simulink model "KUKA_LBR_Simulink_model_flatness_based_control"  (R2017a)
(part 3 of 19)

  cos(q2).*cos(q3).*sin(q1)+cos(q1).*sin(q3))+sin(q1).*sin(q2).*sin(q4))+( ...
  cos(q1).*cos(q3)+(-1).*cos(q2).*sin(q1).*sin(q3)).*sin(q5))+((-1).*cos( ...
  q4).*sin(q1).*sin(q2)+(cos(q2).*cos(q3).*sin(q1)+cos(q1).*sin(q3)).*sin( ...
  q4)).*sin(q6))+(cos(q5).*(cos(q1).*cos(q3)+(-1).*cos(q2).*sin(q1).*sin( ...
  q3))+(-1).*(cos(q4).*(cos(q2).*cos(q3).*sin(q1)+cos(q1).*sin(q3))+sin( ...
  q1).*sin(q2).*sin(q4)).*sin(q5)).*sin(q7)).^2.*(cos(q7).*(cos(q5).*((-1) ...
  .*cos(q3).*sin(q1)+(-1).*cos(q1).*cos(q2).*sin(q3))+(-1).*(cos(q4).*( ...
  cos(q1).*cos(q2).*cos(q3)+(-1).*sin(q1).*sin(q3))+cos(q1).*sin(q2).*sin( ...
  q4)).*sin(q5))+(-1).*(cos(q6).*(cos(q5).*(cos(q4).*(cos(q1).*cos(q2).* ...
  cos(q3)+(-1).*sin(q1).*sin(q3))+cos(q1).*sin(q2).*sin(q4))+((-1).*cos( ...
  q3).*sin(q1)+(-1).*cos(q1).*cos(q2).*sin(q3)).*sin(q5))+((-1).*cos(q1).* ...
  cos(q4).*sin(q2)+(cos(q1).*cos(q2).*cos(q3)+(-1).*sin(q1).*sin(q3)).* ...
  sin(q4)).*sin(q6)).*sin(q7)))+(1+(cos(q7).*(cos(q6).*(cos(q5).*(cos(q4) ...
  .*(cos(q1).*cos(q2).*cos(q3)+(-1).*sin(q1).*sin(q3))+cos(q1).*sin(q2).* ...
  sin(q4))+((-1).*cos(q3).*sin(q1)+(-1).*cos(q1).*cos(q2).*sin(q3)).*sin( ...
  q5))+((-1).*cos(q1).*cos(q4).*sin(q2)+(cos(q1).*cos(q2).*cos(q3)+(-1).* ...
  sin(q1).*sin(q3)).*sin(q4)).*sin(q6))+(cos(q5).*((-1).*cos(q3).*sin(q1)+ ...
  (-1).*cos(q1).*cos(q2).*sin(q3))+(-1).*(cos(q4).*(cos(q1).*cos(q2).*cos( ...
  q3)+(-1).*sin(q1).*sin(q3))+cos(q1).*sin(q2).*sin(q4)).*sin(q5)).*sin( ...
  q7)).^(-2).*(cos(q7).*(cos(q6).*(cos(q5).*(cos(q4).*(cos(q2).*cos(q3).* ...
  sin(q1)+cos(q1).*sin(q3))+sin(q1).*sin(q2).*sin(q4))+(cos(q1).*cos(q3)+( ...
  -1).*cos(q2).*sin(q1).*sin(q3)).*sin(q5))+((-1).*cos(q4).*sin(q1).*sin( ...
  q2)+(cos(q2).*cos(q3).*sin(q1)+cos(q1).*sin(q3)).*sin(q4)).*sin(q6))+( ...
  cos(q5).*(cos(q1).*cos(q3)+(-1).*cos(q2).*sin(q1).*sin(q3))+(-1).*(cos( ...
  q4).*(cos(q2).*cos(q3).*sin(q1)+cos(q1).*sin(q3))+sin(q1).*sin(q2).*sin( ...
  q4)).*sin(q5)).*sin(q7)).^2).^(-1).*((cos(q7).*(cos(q6).*(cos(q5).*(cos( ...
  q4).*(cos(q1).*cos(q2).*cos(q3)+(-1).*sin(q1).*sin(q3))+cos(q1).*sin(q2) ...
  .*sin(q4))+((-1).*cos(q3).*sin(q1)+(-1).*cos(q1).*cos(q2).*sin(q3)).* ...
  sin(q5))+((-1).*cos(q1).*cos(q4).*sin(q2)+(cos(q1).*cos(q2).*cos(q3)+( ...
  -1).*sin(q1).*sin(q3)).*sin(q4)).*sin(q6))+(cos(q5).*((-1).*cos(q3).* ...
  sin(q1)+(-1).*cos(q1).*cos(q2).*sin(q3))+(-1).*(cos(q4).*(cos(q1).*cos( ...
  q2).*cos(q3)+(-1).*sin(q1).*sin(q3))+cos(q1).*sin(q2).*sin(q4)).*sin(q5) ...
  ).*sin(q7)).^(-1).*((-1).*cos(q7).*(cos(q6).*(cos(q5).*(cos(q4).*(cos( ...
  q2).*cos(q3).*sin(q1)+cos(q1).*sin(q3))+sin(q1).*sin(q2).*sin(q4))+(cos( ...
  q1).*cos(q3)+(-1).*cos(q2).*sin(q1).*sin(q3)).*sin(q5))+((-1).*cos(q4).* ...
  sin(q1).*sin(q2)+(cos(q2).*cos(q3).*sin(q1)+cos(q1).*sin(q3)).*sin(q4)) ...
  .*sin(q6))+(-1).*(cos(q5).*(cos(q1).*cos(q3)+(-1).*cos(q2).*sin(q1).* ...
  sin(q3))+(-1).*(cos(q4).*(cos(q2).*cos(q3).*sin(q1)+cos(q1).*sin(q3))+ ...
  sin(q1).*sin(q2).*sin(q4)).*sin(q5)).*sin(q7))+(-1).*((-1).*cos(q7).*( ...
  cos(q6).*(cos(q5).*(cos(q4).*(cos(q1).*cos(q2).*cos(q3)+(-1).*sin(q1).* ...
  sin(q3))+cos(q1).*sin(q2).*sin(q4))+((-1).*cos(q3).*sin(q1)+(-1).*cos( ...
  q1).*cos(q2).*sin(q3)).*sin(q5))+((-1).*cos(q1).*cos(q4).*sin(q2)+(cos( ...
  q1).*cos(q2).*cos(q3)+(-1).*sin(q1).*sin(q3)).*sin(q4)).*sin(q6))+(-1).* ...
  (cos(q5).*((-1).*cos(q3).*sin(q1)+(-1).*cos(q1).*cos(q2).*sin(q3))+(-1) ...
  .*(cos(q4).*(cos(q1).*cos(q2).*cos(q3)+(-1).*sin(q1).*sin(q3))+cos(q1).* ...
  sin(q2).*sin(q4)).*sin(q5)).*sin(q7)).*(cos(q7).*(cos(q6).*(cos(q5).*( ...
  cos(q4).*(cos(q1).*cos(q2).*cos(q3)+(-1).*sin(q1).*sin(q3))+cos(q1).* ...
  sin(q2).*sin(q4))+((-1).*cos(q3).*sin(q1)+(-1).*cos(q1).*cos(q2).*sin( ...
  q3)).*sin(q5))+((-1).*cos(q1).*cos(q4).*sin(q2)+(cos(q1).*cos(q2).*cos( ...
  q3)+(-1).*sin(q1).*sin(q3)).*sin(q4)).*sin(q6))+(cos(q5).*((-1).*cos(q3) ...
  .*sin(q1)+(-1).*cos(q1).*cos(q2).*sin(q3))+(-1).*(cos(q4).*(cos(q1).* ...
  cos(q2).*cos(q3)+(-1).*sin(q1).*sin(q3))+cos(q1).*sin(q2).*sin(q4)).* ...
  sin(q5)).*sin(q7)).^(-2).*(cos(q7).*(cos(q6).*(cos(q5).*(cos(q4).*(cos( ...
  q2).*cos(q3).*sin(q1)+cos(q1).*sin(q3))+sin(q1).*sin(q2).*sin(q4))+(cos( ...
  q1).*cos(q3)+(-1).*cos(q2).*sin(q1).*sin(q3)).*sin(q5))+((-1).*cos(q4).* ...
  sin(q1).*sin(q2)+(cos(q2).*cos(q3).*sin(q1)+cos(q1).*sin(q3)).*sin(q4)) ...
  .*sin(q6))+(cos(q5).*(cos(q1).*cos(q3)+(-1).*cos(q2).*sin(q1).*sin(q3))+ ...
  (-1).*(cos(q4).*(cos(q2).*cos(q3).*sin(q1)+cos(q1).*sin(q3))+sin(q1).* ...
  sin(q2).*sin(q4)).*sin(q5)).*sin(q7))+(-2).*(cos(q7).*(cos(q6).*(cos(q5) ...
  .*(cos(q4).*(cos(q1).*cos(q2).*cos(q3)+(-1).*sin(q1).*sin(q3))+cos(q1).* ...
  sin(q2).*sin(q4))+((-1).*cos(q3).*sin(q1)+(-1).*cos(q1).*cos(q2).*sin( ...
  q3)).*sin(q5))+((-1).*cos(q1).*cos(q4).*sin(q2)+(cos(q1).*cos(q2).*cos( ...
  q3)+(-1).*sin(q1).*sin(q3)).*sin(q4)).*sin(q6))+(cos(q5).*((-1).*cos(q3) ...
  .*sin(q1)+(-1).*cos(q1).*cos(q2).*sin(q3))+(-1).*(cos(q4).*(cos(q1).* ...
  cos(q2).*cos(q3)+(-1).*sin(q1).*sin(q3))+cos(q1).*sin(q2).*sin(q4)).* ...
  sin(q5)).*sin(q7)).^(-2).*(cos(q7).*(cos(q5).*(cos(q1).*cos(q3)+(-1).* ...
  cos(q2).*sin(q1).*sin(q3))+(-1).*(cos(q4).*(cos(q2).*cos(q3).*sin(q1)+ ...
  cos(q1).*sin(q3))+sin(q1).*sin(q2).*sin(q4)).*sin(q5))+(-1).*(cos(q6).*( ...
  cos(q5).*(cos(q4).*(cos(q2).*cos(q3).*sin(q1)+cos(q1).*sin(q3))+sin(q1) ...
  .*sin(q2).*sin(q4))+(cos(q1).*cos(q3)+(-1).*cos(q2).*sin(q1).*sin(q3)).* ...
  sin(q5))+((-1).*cos(q4).*sin(q1).*sin(q2)+(cos(q2).*cos(q3).*sin(q1)+ ...
  cos(q1).*sin(q3)).*sin(q4)).*sin(q6)).*sin(q7)).*(cos(q7).*(cos(q5).*(( ...
  -1).*cos(q3).*sin(q1)+(-1).*cos(q1).*cos(q2).*sin(q3))+(-1).*(cos(q4).*( ...
  cos(q1).*cos(q2).*cos(q3)+(-1).*sin(q1).*sin(q3))+cos(q1).*sin(q2).*sin( ...
  q4)).*sin(q5))+(-1).*(cos(q6).*(cos(q5).*(cos(q4).*(cos(q1).*cos(q2).* ...
  cos(q3)+(-1).*sin(q1).*sin(q3))+cos(q1).*sin(q2).*sin(q4))+((-1).*cos( ...
  q3).*sin(q1)+(-1).*cos(q1).*cos(q2).*sin(q3)).*sin(q5))+((-1).*cos(q1).* ...
  cos(q4).*sin(q2)+(cos(q1).*cos(q2).*cos(q3)+(-1).*sin(q1).*sin(q3)).* ...
  sin(q4)).*sin(q6)).*sin(q7))+2.*(cos(q7).*(cos(q6).*(cos(q5).*(cos(q4).* ...
  (cos(q1).*cos(q2).*cos(q3)+(-1).*sin(q1).*sin(q3))+cos(q1).*sin(q2).* ...
  sin(q4))+((-1).*cos(q3).*sin(q1)+(-1).*cos(q1).*cos(q2).*sin(q3)).*sin( ...
  q5))+((-1).*cos(q1).*cos(q4).*sin(q2)+(cos(q1).*cos(q2).*cos(q3)+(-1).* ...
  sin(q1).*sin(q3)).*sin(q4)).*sin(q6))+(cos(q5).*((-1).*cos(q3).*sin(q1)+ ...
  (-1).*cos(q1).*cos(q2).*sin(q3))+(-1).*(cos(q4).*(cos(q1).*cos(q2).*cos( ...
  q3)+(-1).*sin(q1).*sin(q3))+cos(q1).*sin(q2).*sin(q4)).*sin(q5)).*sin( ...
  q7)).^(-3).*(cos(q7).*(cos(q6).*(cos(q5).*(cos(q4).*(cos(q2).*cos(q3).* ...
  sin(q1)+cos(q1).*sin(q3))+sin(q1).*sin(q2).*sin(q4))+(cos(q1).*cos(q3)+( ...
  -1).*cos(q2).*sin(q1).*sin(q3)).*sin(q5))+((-1).*cos(q4).*sin(q1).*sin( ...
  q2)+(cos(q2).*cos(q3).*sin(q1)+cos(q1).*sin(q3)).*sin(q4)).*sin(q6))+( ...
  cos(q5).*(cos(q1).*cos(q3)+(-1).*cos(q2).*sin(q1).*sin(q3))+(-1).*(cos( ...
  q4).*(cos(q2).*cos(q3).*sin(q1)+cos(q1).*sin(q3))+sin(q1).*sin(q2).*sin( ...
  q4)).*sin(q5)).*sin(q7)).*(cos(q7).*(cos(q5).*((-1).*cos(q3).*sin(q1)+( ...
  -1).*cos(q1).*cos(q2).*sin(q3))+(-1).*(cos(q4).*(cos(q1).*cos(q2).*cos( ...
  q3)+(-1).*sin(q1).*sin(q3))+cos(q1).*sin(q2).*sin(q4)).*sin(q5))+(-1).*( ...
  cos(q6).*(cos(q5).*(cos(q4).*(cos(q1).*cos(q2).*cos(q3)+(-1).*sin(q1).* ...
  sin(q3))+cos(q1).*sin(q2).*sin(q4))+((-1).*cos(q3).*sin(q1)+(-1).*cos( ...
  q1).*cos(q2).*sin(q3)).*sin(q5))+((-1).*cos(q1).*cos(q4).*sin(q2)+(cos( ...
  q1).*cos(q2).*cos(q3)+(-1).*sin(q1).*sin(q3)).*sin(q4)).*sin(q6)).*sin( ...
  q7)).^2);

Jxe251 = 0;

Jxe252 = (-1).*(1+(cos(q7).*(cos(q6).*(cos(q5).*((-1).*cos(q3).*cos( ...
  q4).*sin(q2)+cos(q2).*sin(q4))+sin(q2).*sin(q3).*sin(q5))+((-1).*cos(q2) ...
  .*cos(q4)+(-1).*cos(q3).*sin(q2).*sin(q4)).*sin(q6))+(cos(q5).*sin(q2).* ...
  sin(q3)+(-1).*((-1).*cos(q3).*cos(q4).*sin(q2)+cos(q2).*sin(q4)).*sin( ...
  q5)).*sin(q7)).^2.*(((-1).*cos(q6).*((-1).*cos(q2).*cos(q4)+(-1).*cos( ...
  q3).*sin(q2).*sin(q4))+(cos(q5).*((-1).*cos(q3).*cos(q4).*sin(q2)+cos( ...
  q2).*sin(q4))+sin(q2).*sin(q3).*sin(q5)).*sin(q6)).^2+(cos(q7).*(cos(q5) ...
  .*sin(q2).*sin(q3)+(-1).*((-1).*cos(q3).*cos(q4).*sin(q2)+cos(q2).*sin( ...
  q4)).*sin(q5))+(-1).*(cos(q6).*(cos(q5).*((-1).*cos(q3).*cos(q4).*sin( ...
  q2)+cos(q2).*sin(q4))+sin(q2).*sin(q3).*sin(q5))+((-1).*cos(q2).*cos(q4) ...
  +(-1).*cos(q3).*sin(q2).*sin(q4)).*sin(q6)).*sin(q7)).^2).^(-1)).^(-2).* ...
  ((-1).*(cos(q7).*(cos(q6).*(cos(q5).*((-1).*cos(q3).*cos(q4).*sin(q2)+ ...
  cos(q2).*sin(q4))+sin(q2).*sin(q3).*sin(q5))+((-1).*cos(q2).*cos(q4)+( ...
  -1).*cos(q3).*sin(q2).*sin(q4)).*sin(q6))+(cos(q5).*sin(q2).*sin(q3)+( ...
  -1).*((-1).*cos(q3).*cos(q4).*sin(q2)+cos(q2).*sin(q4)).*sin(q5)).*sin( ...
  q7)).^2.*(2.*((-1).*cos(q6).*(cos(q4).*sin(q2)+(-1).*cos(q2).*cos(q3).* ...
  sin(q4))+(cos(q5).*((-1).*cos(q2).*cos(q3).*cos(q4)+(-1).*sin(q2).*sin( ...
  q4))+cos(q2).*sin(q3).*sin(q5)).*sin(q6)).*((-1).*cos(q6).*((-1).*cos( ...
  q2).*cos(q4)+(-1).*cos(q3).*sin(q2).*sin(q4))+(cos(q5).*((-1).*cos(q3).* ...
  cos(q4).*sin(q2)+cos(q2).*sin(q4))+sin(q2).*sin(q3).*sin(q5)).*sin(q6))+ ...
  2.*(cos(q7).*(cos(q2).*cos(q5).*sin(q3)+(-1).*((-1).*cos(q2).*cos(q3).* ...
  cos(q4)+(-1).*sin(q2).*sin(q4)).*sin(q5))+(-1).*(cos(q6).*(cos(q5).*(( ...
  -1).*cos(q2).*cos(q3).*cos(q4)+(-1).*sin(q2).*sin(q4))+cos(q2).*sin(q3) ...
  .*sin(q5))+(cos(q4).*sin(q2)+(-1).*cos(q2).*cos(q3).*sin(q4)).*sin(q6)) ...
  .*sin(q7)).*(cos(q7).*(cos(q5).*sin(q2).*sin(q3)+(-1).*((-1).*cos(q3).* ...
  cos(q4).*sin(q2)+cos(q2).*sin(q4)).*sin(q5))+(-1).*(cos(q6).*(cos(q5).*( ...
  (-1).*cos(q3).*cos(q4).*sin(q2)+cos(q2).*sin(q4))+sin(q2).*sin(q3).*sin( ...
  q5))+((-1).*cos(q2).*cos(q4)+(-1).*cos(q3).*sin(q2).*sin(q4)).*sin(q6)) ...
  .*sin(q7))).*(((-1).*cos(q6).*((-1).*cos(q2).*cos(q4)+(-1).*cos(q3).* ...
  sin(q2).*sin(q4))+(cos(q5).*((-1).*cos(q3).*cos(q4).*sin(q2)+cos(q2).* ...
  sin(q4))+sin(q2).*sin(q3).*sin(q5)).*sin(q6)).^2+(cos(q7).*(cos(q5).* ...
  sin(q2).*sin(q3)+(-1).*((-1).*cos(q3).*cos(q4).*sin(q2)+cos(q2).*sin(q4) ...
  ).*sin(q5))+(-1).*(cos(q6).*(cos(q5).*((-1).*cos(q3).*cos(q4).*sin(q2)+ ...
  cos(q2).*sin(q4))+sin(q2).*sin(q3).*sin(q5))+((-1).*cos(q2).*cos(q4)+( ...
  -1).*cos(q3).*sin(q2).*sin(q4)).*sin(q6)).*sin(q7)).^2).^(-2)+2.*(cos( ...
  q7).*(cos(q6).*(cos(q5).*((-1).*cos(q3).*cos(q4).*sin(q2)+cos(q2).*sin( ...
  q4))+sin(q2).*sin(q3).*sin(q5))+((-1).*cos(q2).*cos(q4)+(-1).*cos(q3).* ...
  sin(q2).*sin(q4)).*sin(q6))+(cos(q5).*sin(q2).*sin(q3)+(-1).*((-1).*cos( ...
  q3).*cos(q4).*sin(q2)+cos(q2).*sin(q4)).*sin(q5)).*sin(q7)).*(cos(q7).*( ...
  cos(q6).*(cos(q5).*((-1).*cos(q2).*cos(q3).*cos(q4)+(-1).*sin(q2).*sin( ...
  q4))+cos(q2).*sin(q3).*sin(q5))+(cos(q4).*sin(q2)+(-1).*cos(q2).*cos(q3) ...
  .*sin(q4)).*sin(q6))+(cos(q2).*cos(q5).*sin(q3)+(-1).*((-1).*cos(q2).* ...
  cos(q3).*cos(q4)+(-1).*sin(q2).*sin(q4)).*sin(q5)).*sin(q7)).*(((-1).* ...
  cos(q6).*((-1).*cos(q2).*cos(q4)+(-1).*cos(q3).*sin(q2).*sin(q4))+(cos( ...
  q5).*((-1).*cos(q3).*cos(q4).*sin(q2)+cos(q2).*sin(q4))+sin(q2).*sin(q3) ...
  .*sin(q5)).*sin(q6)).^2+(cos(q7).*(cos(q5).*sin(q2).*sin(q3)+(-1).*((-1) ...
  .*cos(q3).*cos(q4).*sin(q2)+cos(q2).*sin(q4)).*sin(q5))+(-1).*(cos(q6).* ...
  (cos(q5).*((-1).*cos(q3).*cos(q4).*sin(q2)+cos(q2).*sin(q4))+sin(q2).* ...
  sin(q3).*sin(q5))+((-1).*cos(q2).*cos(q4)+(-1).*cos(q3).*sin(q2).*sin( ...
  q4)).*sin(q6)).*sin(q7)).^2).^(-1)).*((-1/2).*(cos(q7).*(cos(q6).*(cos( ...
  q5).*((-1).*cos(q3).*cos(q4).*sin(q2)+cos(q2).*sin(q4))+sin(q2).*sin(q3) ...
  .*sin(q5))+((-1).*cos(q2).*cos(q4)+(-1).*cos(q3).*sin(q2).*sin(q4)).* ...
  sin(q6))+(cos(q5).*sin(q2).*sin(q3)+(-1).*((-1).*cos(q3).*cos(q4).*sin( ...
  q2)+cos(q2).*sin(q4)).*sin(q5)).*sin(q7)).*(2.*((-1).*cos(q6).*(cos(q4) ...
  .*sin(q2)+(-1).*cos(q2).*cos(q3).*sin(q4))+(cos(q5).*((-1).*cos(q2).* ...
  cos(q3).*cos(q4)+(-1).*sin(q2).*sin(q4))+cos(q2).*sin(q3).*sin(q5)).* ...
  sin(q6)).*((-1).*cos(q6).*((-1).*cos(q2).*cos(q4)+(-1).*cos(q3).*sin(q2) ...
  .*sin(q4))+(cos(q5).*((-1).*cos(q3).*cos(q4).*sin(q2)+cos(q2).*sin(q4))+ ...
  sin(q2).*sin(q3).*sin(q5)).*sin(q6))+2.*(cos(q7).*(cos(q2).*cos(q5).* ...
  sin(q3)+(-1).*((-1).*cos(q2).*cos(q3).*cos(q4)+(-1).*sin(q2).*sin(q4)).* ...
  sin(q5))+(-1).*(cos(q6).*(cos(q5).*((-1).*cos(q2).*cos(q3).*cos(q4)+(-1) ...
  .*sin(q2).*sin(q4))+cos(q2).*sin(q3).*sin(q5))+(cos(q4).*sin(q2)+(-1).* ...
  cos(q2).*cos(q3).*sin(q4)).*sin(q6)).*sin(q7)).*(cos(q7).*(cos(q5).*sin( ...
  q2).*sin(q3)+(-1).*((-1).*cos(q3).*cos(q4).*sin(q2)+cos(q2).*sin(q4)).* ...
  sin(q5))+(-1).*(cos(q6).*(cos(q5).*((-1).*cos(q3).*cos(q4).*sin(q2)+cos( ...
  q2).*sin(q4))+sin(q2).*sin(q3).*sin(q5))+((-1).*cos(q2).*cos(q4)+(-1).* ...
  cos(q3).*sin(q2).*sin(q4)).*sin(q6)).*sin(q7))).*(((-1).*cos(q6).*((-1) ...
  .*cos(q2).*cos(q4)+(-1).*cos(q3).*sin(q2).*sin(q4))+(cos(q5).*((-1).* ...
  cos(q3).*cos(q4).*sin(q2)+cos(q2).*sin(q4))+sin(q2).*sin(q3).*sin(q5)).* ...
  sin(q6)).^2+(cos(q7).*(cos(q5).*sin(q2).*sin(q3)+(-1).*((-1).*cos(q3).* ...
  cos(q4).*sin(q2)+cos(q2).*sin(q4)).*sin(q5))+(-1).*(cos(q6).*(cos(q5).*( ...
  (-1).*cos(q3).*cos(q4).*sin(q2)+cos(q2).*sin(q4))+sin(q2).*sin(q3).*sin( ...
  q5))+((-1).*cos(q2).*cos(q4)+(-1).*cos(q3).*sin(q2).*sin(q4)).*sin(q6)) ...
  .*sin(q7)).^2).^(-3/2)+(cos(q7).*(cos(q6).*(cos(q5).*((-1).*cos(q2).* ...
  cos(q3).*cos(q4)+(-1).*sin(q2).*sin(q4))+cos(q2).*sin(q3).*sin(q5))+( ...
  cos(q4).*sin(q2)+(-1).*cos(q2).*cos(q3).*sin(q4)).*sin(q6))+(cos(q2).* ...
  cos(q5).*sin(q3)+(-1).*((-1).*cos(q2).*cos(q3).*cos(q4)+(-1).*sin(q2).* ...
  sin(q4)).*sin(q5)).*sin(q7)).*(((-1).*cos(q6).*((-1).*cos(q2).*cos(q4)+( ...
  -1).*cos(q3).*sin(q2).*sin(q4))+(cos(q5).*((-1).*cos(q3).*cos(q4).*sin( ...
  q2)+cos(q2).*sin(q4))+sin(q2).*sin(q3).*sin(q5)).*sin(q6)).^2+(cos(q7).* ...
  (cos(q5).*sin(q2).*sin(q3)+(-1).*((-1).*cos(q3).*cos(q4).*sin(q2)+cos( ...
  q2).*sin(q4)).*sin(q5))+(-1).*(cos(q6).*(cos(q5).*((-1).*cos(q3).*cos( ...
  q4).*sin(q2)+cos(q2).*sin(q4))+sin(q2).*sin(q3).*sin(q5))+((-1).*cos(q2) ...
  .*cos(q4)+(-1).*cos(q3).*sin(q2).*sin(q4)).*sin(q6)).*sin(q7)).^2).^( ...
  -1/2))+(1+(cos(q7).*(cos(q6).*(cos(q5).*((-1).*cos(q3).*cos(q4).*sin(q2) ...
  +cos(q2).*sin(q4))+sin(q2).*sin(q3).*sin(q5))+((-1).*cos(q2).*cos(q4)+( ...
  -1).*cos(q3).*sin(q2).*sin(q4)).*sin(q6))+(cos(q5).*sin(q2).*sin(q3)+( ...
  -1).*((-1).*cos(q3).*cos(q4).*sin(q2)+cos(q2).*sin(q4)).*sin(q5)).*sin( ...
  q7)).^2.*(((-1).*cos(q6).*((-1).*cos(q2).*cos(q4)+(-1).*cos(q3).*sin(q2) ...
  .*sin(q4))+(cos(q5).*((-1).*cos(q3).*cos(q4).*sin(q2)+cos(q2).*sin(q4))+ ...
  sin(q2).*sin(q3).*sin(q5)).*sin(q6)).^2+(cos(q7).*(cos(q5).*sin(q2).* ...
  sin(q3)+(-1).*((-1).*cos(q3).*cos(q4).*sin(q2)+cos(q2).*sin(q4)).*sin( ...
  q5))+(-1).*(cos(q6).*(cos(q5).*((-1).*cos(q3).*cos(q4).*sin(q2)+cos(q2) ...
  .*sin(q4))+sin(q2).*sin(q3).*sin(q5))+((-1).*cos(q2).*cos(q4)+(-1).*cos( ...
  q3).*sin(q2).*sin(q4)).*sin(q6)).*sin(q7)).^2).^(-1)).^(-1).*((3/4).*( ...
  cos(q7).*(cos(q6).*(cos(q5).*((-1).*cos(q3).*cos(q4).*sin(q2)+cos(q2).* ...
  sin(q4))+sin(q2).*sin(q3).*sin(q5))+((-1).*cos(q2).*cos(q4)+(-1).*cos( ...
  q3).*sin(q2).*sin(q4)).*sin(q6))+(cos(q5).*sin(q2).*sin(q3)+(-1).*((-1) ...
  .*cos(q3).*cos(q4).*sin(q2)+cos(q2).*sin(q4)).*sin(q5)).*sin(q7)).*(2.*( ...
  (-1).*cos(q6).*(cos(q4).*sin(q2)+(-1).*cos(q2).*cos(q3).*sin(q4))+(cos( ...
  q5).*((-1).*cos(q2).*cos(q3).*cos(q4)+(-1).*sin(q2).*sin(q4))+cos(q2).* ...
  sin(q3).*sin(q5)).*sin(q6)).*((-1).*cos(q6).*((-1).*cos(q2).*cos(q4)+( ...
  -1).*cos(q3).*sin(q2).*sin(q4))+(cos(q5).*((-1).*cos(q3).*cos(q4).*sin( ...
  q2)+cos(q2).*sin(q4))+sin(q2).*sin(q3).*sin(q5)).*sin(q6))+2.*(cos(q7).* ...
  (cos(q2).*cos(q5).*sin(q3)+(-1).*((-1).*cos(q2).*cos(q3).*cos(q4)+(-1).* ...
  sin(q2).*sin(q4)).*sin(q5))+(-1).*(cos(q6).*(cos(q5).*((-1).*cos(q2).* ...
  cos(q3).*cos(q4)+(-1).*sin(q2).*sin(q4))+cos(q2).*sin(q3).*sin(q5))+( ...
  cos(q4).*sin(q2)+(-1).*cos(q2).*cos(q3).*sin(q4)).*sin(q6)).*sin(q7)).*( ...
  cos(q7).*(cos(q5).*sin(q2).*sin(q3)+(-1).*((-1).*cos(q3).*cos(q4).*sin( ...
  q2)+cos(q2).*sin(q4)).*sin(q5))+(-1).*(cos(q6).*(cos(q5).*((-1).*cos(q3) ...
  .*cos(q4).*sin(q2)+cos(q2).*sin(q4))+sin(q2).*sin(q3).*sin(q5))+((-1).* ...
  cos(q2).*cos(q4)+(-1).*cos(q3).*sin(q2).*sin(q4)).*sin(q6)).*sin(q7))) ...
  .^2.*(((-1).*cos(q6).*((-1).*cos(q2).*cos(q4)+(-1).*cos(q3).*sin(q2).* ...
  sin(q4))+(cos(q5).*((-1).*cos(q3).*cos(q4).*sin(q2)+cos(q2).*sin(q4))+ ...
  sin(q2).*sin(q3).*sin(q5)).*sin(q6)).^2+(cos(q7).*(cos(q5).*sin(q2).* ...
  sin(q3)+(-1).*((-1).*cos(q3).*cos(q4).*sin(q2)+cos(q2).*sin(q4)).*sin( ...
  q5))+(-1).*(cos(q6).*(cos(q5).*((-1).*cos(q3).*cos(q4).*sin(q2)+cos(q2) ...
  .*sin(q4))+sin(q2).*sin(q3).*sin(q5))+((-1).*cos(q2).*cos(q4)+(-1).*cos( ...
  q3).*sin(q2).*sin(q4)).*sin(q6)).*sin(q7)).^2).^(-5/2)+(-1).*(cos(q7).*( ...
  cos(q6).*(cos(q5).*((-1).*cos(q2).*cos(q3).*cos(q4)+(-1).*sin(q2).*sin( ...
  q4))+cos(q2).*sin(q3).*sin(q5))+(cos(q4).*sin(q2)+(-1).*cos(q2).*cos(q3) ...
  .*sin(q4)).*sin(q6))+(cos(q2).*cos(q5).*sin(q3)+(-1).*((-1).*cos(q2).* ...
  cos(q3).*cos(q4)+(-1).*sin(q2).*sin(q4)).*sin(q5)).*sin(q7)).*(2.*((-1) ...
  .*cos(q6).*(cos(q4).*sin(q2)+(-1).*cos(q2).*cos(q3).*sin(q4))+(cos(q5).* ...
  ((-1).*cos(q2).*cos(q3).*cos(q4)+(-1).*sin(q2).*sin(q4))+cos(q2).*sin( ...
  q3).*sin(q5)).*sin(q6)).*((-1).*cos(q6).*((-1).*cos(q2).*cos(q4)+(-1).* ...
  cos(q3).*sin(q2).*sin(q4))+(cos(q5).*((-1).*cos(q3).*cos(q4).*sin(q2)+ ...
  cos(q2).*sin(q4))+sin(q2).*sin(q3).*sin(q5)).*sin(q6))+2.*(cos(q7).*( ...
  cos(q2).*cos(q5).*sin(q3)+(-1).*((-1).*cos(q2).*cos(q3).*cos(q4)+(-1).* ...
  sin(q2).*sin(q4)).*sin(q5))+(-1).*(cos(q6).*(cos(q5).*((-1).*cos(q2).* ...
  cos(q3).*cos(q4)+(-1).*sin(q2).*sin(q4))+cos(q2).*sin(q3).*sin(q5))+( ...
  cos(q4).*sin(q2)+(-1).*cos(q2).*cos(q3).*sin(q4)).*sin(q6)).*sin(q7)).*( ...
  cos(q7).*(cos(q5).*sin(q2).*sin(q3)+(-1).*((-1).*cos(q3).*cos(q4).*sin( ...
  q2)+cos(q2).*sin(q4)).*sin(q5))+(-1).*(cos(q6).*(cos(q5).*((-1).*cos(q3) ...
  .*cos(q4).*sin(q2)+cos(q2).*sin(q4))+sin(q2).*sin(q3).*sin(q5))+((-1).* ...
  cos(q2).*cos(q4)+(-1).*cos(q3).*sin(q2).*sin(q4)).*sin(q6)).*sin(q7))).* ...
  (((-1).*cos(q6).*((-1).*cos(q2).*cos(q4)+(-1).*cos(q3).*sin(q2).*sin(q4) ...
  )+(cos(q5).*((-1).*cos(q3).*cos(q4).*sin(q2)+cos(q2).*sin(q4))+sin(q2).* ...
  sin(q3).*sin(q5)).*sin(q6)).^2+(cos(q7).*(cos(q5).*sin(q2).*sin(q3)+(-1) ...
  .*((-1).*cos(q3).*cos(q4).*sin(q2)+cos(q2).*sin(q4)).*sin(q5))+(-1).*( ...
  cos(q6).*(cos(q5).*((-1).*cos(q3).*cos(q4).*sin(q2)+cos(q2).*sin(q4))+ ...
  sin(q2).*sin(q3).*sin(q5))+((-1).*cos(q2).*cos(q4)+(-1).*cos(q3).*sin( ...
  q2).*sin(q4)).*sin(q6)).*sin(q7)).^2).^(-3/2)+(cos(q7).*(cos(q6).*(cos( ...
  q5).*(cos(q3).*cos(q4).*sin(q2)+(-1).*cos(q2).*sin(q4))+(-1).*sin(q2).* ...
  sin(q3).*sin(q5))+(cos(q2).*cos(q4)+cos(q3).*sin(q2).*sin(q4)).*sin(q6)) ...
  +((-1).*cos(q5).*sin(q2).*sin(q3)+(-1).*(cos(q3).*cos(q4).*sin(q2)+(-1) ...
  .*cos(q2).*sin(q4)).*sin(q5)).*sin(q7)).*(((-1).*cos(q6).*((-1).*cos(q2) ...
  .*cos(q4)+(-1).*cos(q3).*sin(q2).*sin(q4))+(cos(q5).*((-1).*cos(q3).* ...
  cos(q4).*sin(q2)+cos(q2).*sin(q4))+sin(q2).*sin(q3).*sin(q5)).*sin(q6)) ...
  .^2+(cos(q7).*(cos(q5).*sin(q2).*sin(q3)+(-1).*((-1).*cos(q3).*cos(q4).* ...
  sin(q2)+cos(q2).*sin(q4)).*sin(q5))+(-1).*(cos(q6).*(cos(q5).*((-1).* ...
  cos(q3).*cos(q4).*sin(q2)+cos(q2).*sin(q4))+sin(q2).*sin(q3).*sin(q5))+( ...
  (-1).*cos(q2).*cos(q4)+(-1).*cos(q3).*sin(q2).*sin(q4)).*sin(q6)).*sin( ...
  q7)).^2).^(-1/2)+(-1/2).*(cos(q7).*(cos(q6).*(cos(q5).*((-1).*cos(q3).* ...
  cos(q4).*sin(q2)+cos(q2).*sin(q4))+sin(q2).*sin(q3).*sin(q5))+((-1).* ...
  cos(q2).*cos(q4)+(-1).*cos(q3).*sin(q2).*sin(q4)).*sin(q6))+(cos(q5).* ...
  sin(q2).*sin(q3)+(-1).*((-1).*cos(q3).*cos(q4).*sin(q2)+cos(q2).*sin(q4) ...
  ).*sin(q5)).*sin(q7)).*(((-1).*cos(q6).*((-1).*cos(q2).*cos(q4)+(-1).* ...
  cos(q3).*sin(q2).*sin(q4))+(cos(q5).*((-1).*cos(q3).*cos(q4).*sin(q2)+ ...
  cos(q2).*sin(q4))+sin(q2).*sin(q3).*sin(q5)).*sin(q6)).^2+(cos(q7).*( ...
  cos(q5).*sin(q2).*sin(q3)+(-1).*((-1).*cos(q3).*cos(q4).*sin(q2)+cos(q2) ...
  .*sin(q4)).*sin(q5))+(-1).*(cos(q6).*(cos(q5).*((-1).*cos(q3).*cos(q4).* ...
  sin(q2)+cos(q2).*sin(q4))+sin(q2).*sin(q3).*sin(q5))+((-1).*cos(q2).* ...
  cos(q4)+(-1).*cos(q3).*sin(q2).*sin(q4)).*sin(q6)).*sin(q7)).^2).^(-3/2) ...
  .*(2.*((-1).*cos(q6).*(cos(q4).*sin(q2)+(-1).*cos(q2).*cos(q3).*sin(q4)) ...
  +(cos(q5).*((-1).*cos(q2).*cos(q3).*cos(q4)+(-1).*sin(q2).*sin(q4))+cos( ...
  q2).*sin(q3).*sin(q5)).*sin(q6)).^2+2.*((-1).*cos(q6).*(cos(q2).*cos(q4) ...
  +cos(q3).*sin(q2).*sin(q4))+(cos(q5).*(cos(q3).*cos(q4).*sin(q2)+(-1).* ...
  cos(q2).*sin(q4))+(-1).*sin(q2).*sin(q3).*sin(q5)).*sin(q6)).*((-1).* ...
  cos(q6).*((-1).*cos(q2).*cos(q4)+(-1).*cos(q3).*sin(q2).*sin(q4))+(cos( ...
  q5).*((-1).*cos(q3).*cos(q4).*sin(q2)+cos(q2).*sin(q4))+sin(q2).*sin(q3) ...
  .*sin(q5)).*sin(q6))+2.*(cos(q7).*(cos(q2).*cos(q5).*sin(q3)+(-1).*((-1) ...
  .*cos(q2).*cos(q3).*cos(q4)+(-1).*sin(q2).*sin(q4)).*sin(q5))+(-1).*( ...
  cos(q6).*(cos(q5).*((-1).*cos(q2).*cos(q3).*cos(q4)+(-1).*sin(q2).*sin( ...
  q4))+cos(q2).*sin(q3).*sin(q5))+(cos(q4).*sin(q2)+(-1).*cos(q2).*cos(q3) ...
  .*sin(q4)).*sin(q6)).*sin(q7)).^2+2.*(cos(q7).*(cos(q5).*sin(q2).*sin( ...
  q3)+(-1).*((-1).*cos(q3).*cos(q4).*sin(q2)+cos(q2).*sin(q4)).*sin(q5))+( ...
  -1).*(cos(q6).*(cos(q5).*((-1).*cos(q3).*cos(q4).*sin(q2)+cos(q2).*sin( ...
  q4))+sin(q2).*sin(q3).*sin(q5))+((-1).*cos(q2).*cos(q4)+(-1).*cos(q3).* ...
  sin(q2).*sin(q4)).*sin(q6)).*sin(q7)).*(cos(q7).*((-1).*cos(q5).*sin(q2) ...
  .*sin(q3)+(-1).*(cos(q3).*cos(q4).*sin(q2)+(-1).*cos(q2).*sin(q4)).*sin( ...
  q5))+(-1).*(cos(q6).*(cos(q5).*(cos(q3).*cos(q4).*sin(q2)+(-1).*cos(q2) ...
  .*sin(q4))+(-1).*sin(q2).*sin(q3).*sin(q5))+(cos(q2).*cos(q4)+cos(q3).* ...
  sin(q2).*sin(q4)).*sin(q6)).*sin(q7))));

Jxe253 = (1+(cos(q7).*(cos(q6).*(cos(q5) ...
  .*((-1).*cos(q3).*cos(q4).*sin(q2)+cos(q2).*sin(q4))+sin(q2).*sin(q3).* ...
  sin(q5))+((-1).*cos(q2).*cos(q4)+(-1).*cos(q3).*sin(q2).*sin(q4)).*sin( ...
  q6))+(cos(q5).*sin(q2).*sin(q3)+(-1).*((-1).*cos(q3).*cos(q4).*sin(q2)+ ...
  cos(q2).*sin(q4)).*sin(q5)).*sin(q7)).^2.*(((-1).*cos(q6).*((-1).*cos( ...
  q2).*cos(q4)+(-1).*cos(q3).*sin(q2).*sin(q4))+(cos(q5).*((-1).*cos(q3).* ...
  cos(q4).*sin(q2)+cos(q2).*sin(q4))+sin(q2).*sin(q3).*sin(q5)).*sin(q6)) ...
  .^2+(cos(q7).*(cos(q5).*sin(q2).*sin(q3)+(-1).*((-1).*cos(q3).*cos(q4).* ...
  sin(q2)+cos(q2).*sin(q4)).*sin(q5))+(-1).*(cos(q6).*(cos(q5).*((-1).* ...
  cos(q3).*cos(q4).*sin(q2)+cos(q2).*sin(q4))+sin(q2).*sin(q3).*sin(q5))+( ...
  (-1).*cos(q2).*cos(q4)+(-1).*cos(q3).*sin(q2).*sin(q4)).*sin(q6)).*sin( ...
  q7)).^2).^(-1)).^(-1).*((3/4).*(cos(q7).*(cos(q6).*(cos(q5).*((-1).*cos( ...
  q3).*cos(q4).*sin(q2)+cos(q2).*sin(q4))+sin(q2).*sin(q3).*sin(q5))+((-1) ...
  .*cos(q2).*cos(q4)+(-1).*cos(q3).*sin(q2).*sin(q4)).*sin(q6))+(cos(q5).* ...
  sin(q2).*sin(q3)+(-1).*((-1).*cos(q3).*cos(q4).*sin(q2)+cos(q2).*sin(q4) ...
  ).*sin(q5)).*sin(q7)).*(2.*((-1).*cos(q6).*sin(q2).*sin(q3).*sin(q4)+( ...
  cos(q4).*cos(q5).*sin(q2).*sin(q3)+cos(q3).*sin(q2).*sin(q5)).*sin(q6)) ...
  .*((-1).*cos(q6).*((-1).*cos(q2).*cos(q4)+(-1).*cos(q3).*sin(q2).*sin( ...
  q4))+(cos(q5).*((-1).*cos(q3).*cos(q4).*sin(q2)+cos(q2).*sin(q4))+sin( ...
  q2).*sin(q3).*sin(q5)).*sin(q6))+2.*(cos(q7).*(cos(q3).*cos(q5).*sin(q2) ...
  +(-1).*cos(q4).*sin(q2).*sin(q3).*sin(q5))+(-1).*(cos(q6).*(cos(q4).* ...
  cos(q5).*sin(q2).*sin(q3)+cos(q3).*sin(q2).*sin(q5))+sin(q2).*sin(q3).* ...
  sin(q4).*sin(q6)).*sin(q7)).*(cos(q7).*(cos(q5).*sin(q2).*sin(q3)+(-1).* ...
  ((-1).*cos(q3).*cos(q4).*sin(q2)+cos(q2).*sin(q4)).*sin(q5))+(-1).*(cos( ...
  q6).*(cos(q5).*((-1).*cos(q3).*cos(q4).*sin(q2)+cos(q2).*sin(q4))+sin( ...
  q2).*sin(q3).*sin(q5))+((-1).*cos(q2).*cos(q4)+(-1).*cos(q3).*sin(q2).* ...
  sin(q4)).*sin(q6)).*sin(q7))).^2.*(((-1).*cos(q6).*((-1).*cos(q2).*cos( ...
  q4)+(-1).*cos(q3).*sin(q2).*sin(q4))+(cos(q5).*((-1).*cos(q3).*cos(q4).* ...
  sin(q2)+cos(q2).*sin(q4))+sin(q2).*sin(q3).*sin(q5)).*sin(q6)).^2+(cos( ...
  q7).*(cos(q5).*sin(q2).*sin(q3)+(-1).*((-1).*cos(q3).*cos(q4).*sin(q2)+ ...
  cos(q2).*sin(q4)).*sin(q5))+(-1).*(cos(q6).*(cos(q5).*((-1).*cos(q3).* ...
  cos(q4).*sin(q2)+cos(q2).*sin(q4))+sin(q2).*sin(q3).*sin(q5))+((-1).* ...
  cos(q2).*cos(q4)+(-1).*cos(q3).*sin(q2).*sin(q4)).*sin(q6)).*sin(q7)) ...
  .^2).^(-5/2)+(-1/2).*(cos(q7).*(cos(q6).*(cos(q5).*((-1).*cos(q3).*cos( ...
  q4).*sin(q2)+cos(q2).*sin(q4))+sin(q2).*sin(q3).*sin(q5))+((-1).*cos(q2) ...
  .*cos(q4)+(-1).*cos(q3).*sin(q2).*sin(q4)).*sin(q6))+(cos(q5).*sin(q2).* ...
  sin(q3)+(-1).*((-1).*cos(q3).*cos(q4).*sin(q2)+cos(q2).*sin(q4)).*sin( ...
  q5)).*sin(q7)).*(2.*((-1).*cos(q6).*sin(q2).*sin(q3).*sin(q4)+(cos(q4).* ...
  cos(q5).*sin(q2).*sin(q3)+cos(q3).*sin(q2).*sin(q5)).*sin(q6)).^2+2.*(( ...
  -1).*cos(q3).*cos(q6).*sin(q2).*sin(q4)+(cos(q3).*cos(q4).*cos(q5).*sin( ...
  q2)+(-1).*sin(q2).*sin(q3).*sin(q5)).*sin(q6)).*((-1).*cos(q6).*((-1).* ...
  cos(q2).*cos(q4)+(-1).*cos(q3).*sin(q2).*sin(q4))+(cos(q5).*((-1).*cos( ...
  q3).*cos(q4).*sin(q2)+cos(q2).*sin(q4))+sin(q2).*sin(q3).*sin(q5)).*sin( ...
  q6))+2.*(cos(q7).*(cos(q3).*cos(q5).*sin(q2)+(-1).*cos(q4).*sin(q2).* ...
  sin(q3).*sin(q5))+(-1).*(cos(q6).*(cos(q4).*cos(q5).*sin(q2).*sin(q3)+ ...
  cos(q3).*sin(q2).*sin(q5))+sin(q2).*sin(q3).*sin(q4).*sin(q6)).*sin(q7)) ...
  .^2+2.*(cos(q7).*((-1).*cos(q5).*sin(q2).*sin(q3)+(-1).*cos(q3).*cos(q4) ...
  .*sin(q2).*sin(q5))+(-1).*(cos(q6).*(cos(q3).*cos(q4).*cos(q5).*sin(q2)+ ...
  (-1).*sin(q2).*sin(q3).*sin(q5))+cos(q3).*sin(q2).*sin(q4).*sin(q6)).* ...
  sin(q7)).*(cos(q7).*(cos(q5).*sin(q2).*sin(q3)+(-1).*((-1).*cos(q3).* ...
  cos(q4).*sin(q2)+cos(q2).*sin(q4)).*sin(q5))+(-1).*(cos(q6).*(cos(q5).*( ...
  (-1).*cos(q3).*cos(q4).*sin(q2)+cos(q2).*sin(q4))+sin(q2).*sin(q3).*sin( ...
  q5))+((-1).*cos(q2).*cos(q4)+(-1).*cos(q3).*sin(q2).*sin(q4)).*sin(q6)) ...
  .*sin(q7))).*(((-1).*cos(q6).*((-1).*cos(q2).*cos(q4)+(-1).*cos(q3).* ...
  sin(q2).*sin(q4))+(cos(q5).*((-1).*cos(q3).*cos(q4).*sin(q2)+cos(q2).* ...
  sin(q4))+sin(q2).*sin(q3).*sin(q5)).*sin(q6)).^2+(cos(q7).*(cos(q5).* ...
  sin(q2).*sin(q3)+(-1).*((-1).*cos(q3).*cos(q4).*sin(q2)+cos(q2).*sin(q4) ...
  ).*sin(q5))+(-1).*(cos(q6).*(cos(q5).*((-1).*cos(q3).*cos(q4).*sin(q2)+ ...
  cos(q2).*sin(q4))+sin(q2).*sin(q3).*sin(q5))+((-1).*cos(q2).*cos(q4)+( ...
  -1).*cos(q3).*sin(q2).*sin(q4)).*sin(q6)).*sin(q7)).^2).^(-3/2)+(-1).*( ...
  cos(q7).*(cos(q6).*(cos(q4).*cos(q5).*sin(q2).*sin(q3)+cos(q3).*sin(q2) ...
  .*sin(q5))+sin(q2).*sin(q3).*sin(q4).*sin(q6))+(cos(q3).*cos(q5).*sin( ...
  q2)+(-1).*cos(q4).*sin(q2).*sin(q3).*sin(q5)).*sin(q7)).*(2.*((-1).*cos( ...
  q6).*sin(q2).*sin(q3).*sin(q4)+(cos(q4).*cos(q5).*sin(q2).*sin(q3)+cos( ...
  q3).*sin(q2).*sin(q5)).*sin(q6)).*((-1).*cos(q6).*((-1).*cos(q2).*cos( ...
  q4)+(-1).*cos(q3).*sin(q2).*sin(q4))+(cos(q5).*((-1).*cos(q3).*cos(q4).* ...
  sin(q2)+cos(q2).*sin(q4))+sin(q2).*sin(q3).*sin(q5)).*sin(q6))+2.*(cos( ...
  q7).*(cos(q3).*cos(q5).*sin(q2)+(-1).*cos(q4).*sin(q2).*sin(q3).*sin(q5) ...
  )+(-1).*(cos(q6).*(cos(q4).*cos(q5).*sin(q2).*sin(q3)+cos(q3).*sin(q2).* ...
  sin(q5))+sin(q2).*sin(q3).*sin(q4).*sin(q6)).*sin(q7)).*(cos(q7).*(cos( ...
  q5).*sin(q2).*sin(q3)+(-1).*((-1).*cos(q3).*cos(q4).*sin(q2)+cos(q2).* ...
  sin(q4)).*sin(q5))+(-1).*(cos(q6).*(cos(q5).*((-1).*cos(q3).*cos(q4).* ...
  sin(q2)+cos(q2).*sin(q4))+sin(q2).*sin(q3).*sin(q5))+((-1).*cos(q2).* ...
  cos(q4)+(-1).*cos(q3).*sin(q2).*sin(q4)).*sin(q6)).*sin(q7))).*(((-1).* ...
  cos(q6).*((-1).*cos(q2).*cos(q4)+(-1).*cos(q3).*sin(q2).*sin(q4))+(cos( ...
  q5).*((-1).*cos(q3).*cos(q4).*sin(q2)+cos(q2).*sin(q4))+sin(q2).*sin(q3) ...
  .*sin(q5)).*sin(q6)).^2+(cos(q7).*(cos(q5).*sin(q2).*sin(q3)+(-1).*((-1) ...
  .*cos(q3).*cos(q4).*sin(q2)+cos(q2).*sin(q4)).*sin(q5))+(-1).*(cos(q6).* ...
  (cos(q5).*((-1).*cos(q3).*cos(q4).*sin(q2)+cos(q2).*sin(q4))+sin(q2).* ...
  sin(q3).*sin(q5))+((-1).*cos(q2).*cos(q4)+(-1).*cos(q3).*sin(q2).*sin( ...
  q4)).*sin(q6)).*sin(q7)).^2).^(-3/2)+(cos(q7).*(cos(q6).*(cos(q3).*cos( ...
  q4).*cos(q5).*sin(q2)+(-1).*sin(q2).*sin(q3).*sin(q5))+cos(q3).*sin(q2) ...
  .*sin(q4).*sin(q6))+((-1).*cos(q5).*sin(q2).*sin(q3)+(-1).*cos(q3).*cos( ...
  q4).*sin(q2).*sin(q5)).*sin(q7)).*(((-1).*cos(q6).*((-1).*cos(q2).*cos( ...
  q4)+(-1).*cos(q3).*sin(q2).*sin(q4))+(cos(q5).*((-1).*cos(q3).*cos(q4).* ...
  sin(q2)+cos(q2).*sin(q4))+sin(q2).*sin(q3).*sin(q5)).*sin(q6)).^2+(cos( ...
  q7).*(cos(q5).*sin(q2).*sin(q3)+(-1).*((-1).*cos(q3).*cos(q4).*sin(q2)+ ...
  cos(q2).*sin(q4)).*sin(q5))+(-1).*(cos(q6).*(cos(q5).*((-1).*cos(q3).* ...
  cos(q4).*sin(q2)+cos(q2).*sin(q4))+sin(q2).*sin(q3).*sin(q5))+((-1).* ...
  cos(q2).*cos(q4)+(-1).*cos(q3).*sin(q2).*sin(q4)).*sin(q6)).*sin(q7)) ...
  .^2).^(-1/2))+(-1).*((-1).*(cos(q7).*(cos(q6).*(cos(q5).*((-1).*cos(q3) ...
  .*cos(q4).*sin(q2)+cos(q2).*sin(q4))+sin(q2).*sin(q3).*sin(q5))+((-1).* ...
  cos(q2).*cos(q4)+(-1).*cos(q3).*sin(q2).*sin(q4)).*sin(q6))+(cos(q5).* ...
  sin(q2).*sin(q3)+(-1).*((-1).*cos(q3).*cos(q4).*sin(q2)+cos(q2).*sin(q4) ...
  ).*sin(q5)).*sin(q7)).^2.*(2.*((-1).*cos(q6).*sin(q2).*sin(q3).*sin(q4)+ ...
  (cos(q4).*cos(q5).*sin(q2).*sin(q3)+cos(q3).*sin(q2).*sin(q5)).*sin(q6)) ...
  .*((-1).*cos(q6).*((-1).*cos(q2).*cos(q4)+(-1).*cos(q3).*sin(q2).*sin( ...
  q4))+(cos(q5).*((-1).*cos(q3).*cos(q4).*sin(q2)+cos(q2).*sin(q4))+sin( ...
  q2).*sin(q3).*sin(q5)).*sin(q6))+2.*(cos(q7).*(cos(q3).*cos(q5).*sin(q2) ...
  +(-1).*cos(q4).*sin(q2).*sin(q3).*sin(q5))+(-1).*(cos(q6).*(cos(q4).* ...
  cos(q5).*sin(q2).*sin(q3)+cos(q3).*sin(q2).*sin(q5))+sin(q2).*sin(q3).* ...
  sin(q4).*sin(q6)).*sin(q7)).*(cos(q7).*(cos(q5).*sin(q2).*sin(q3)+(-1).* ...
  ((-1).*cos(q3).*cos(q4).*sin(q2)+cos(q2).*sin(q4)).*sin(q5))+(-1).*(cos( ...
  q6).*(cos(q5).*((-1).*cos(q3).*cos(q4).*sin(q2)+cos(q2).*sin(q4))+sin( ...
  q2).*sin(q3).*sin(q5))+((-1).*cos(q2).*cos(q4)+(-1).*cos(q3).*sin(q2).* ...
  sin(q4)).*sin(q6)).*sin(q7))).*(((-1).*cos(q6).*((-1).*cos(q2).*cos(q4)+ ...
  (-1).*cos(q3).*sin(q2).*sin(q4))+(cos(q5).*((-1).*cos(q3).*cos(q4).*sin( ...
  q2)+cos(q2).*sin(q4))+sin(q2).*sin(q3).*sin(q5)).*sin(q6)).^2+(cos(q7).* ...
  (cos(q5).*sin(q2).*sin(q3)+(-1).*((-1).*cos(q3).*cos(q4).*sin(q2)+cos( ...
  q2).*sin(q4)).*sin(q5))+(-1).*(cos(q6).*(cos(q5).*((-1).*cos(q3).*cos( ...
  q4).*sin(q2)+cos(q2).*sin(q4))+sin(q2).*sin(q3).*sin(q5))+((-1).*cos(q2) ...
  .*cos(q4)+(-1).*cos(q3).*sin(q2).*sin(q4)).*sin(q6)).*sin(q7)).^2).^(-2) ...
  +2.*(cos(q7).*(cos(q6).*(cos(q4).*cos(q5).*sin(q2).*sin(q3)+cos(q3).* ...
  sin(q2).*sin(q5))+sin(q2).*sin(q3).*sin(q4).*sin(q6))+(cos(q3).*cos(q5) ...
  .*sin(q2)+(-1).*cos(q4).*sin(q2).*sin(q3).*sin(q5)).*sin(q7)).*(cos(q7) ...
  .*(cos(q6).*(cos(q5).*((-1).*cos(q3).*cos(q4).*sin(q2)+cos(q2).*sin(q4)) ...
  +sin(q2).*sin(q3).*sin(q5))+((-1).*cos(q2).*cos(q4)+(-1).*cos(q3).*sin( ...
  q2).*sin(q4)).*sin(q6))+(cos(q5).*sin(q2).*sin(q3)+(-1).*((-1).*cos(q3) ...
  .*cos(q4).*sin(q2)+cos(q2).*sin(q4)).*sin(q5)).*sin(q7)).*(((-1).*cos( ...
  q6).*((-1).*cos(q2).*cos(q4)+(-1).*cos(q3).*sin(q2).*sin(q4))+(cos(q5).* ...
  ((-1).*cos(q3).*cos(q4).*sin(q2)+cos(q2).*sin(q4))+sin(q2).*sin(q3).* ...
  sin(q5)).*sin(q6)).^2+(cos(q7).*(cos(q5).*sin(q2).*sin(q3)+(-1).*((-1).* ...
  cos(q3).*cos(q4).*sin(q2)+cos(q2).*sin(q4)).*sin(q5))+(-1).*(cos(q6).*( ...
  cos(q5).*((-1).*cos(q3).*cos(q4).*sin(q2)+cos(q2).*sin(q4))+sin(q2).* ...
  sin(q3).*sin(q5))+((-1).*cos(q2).*cos(q4)+(-1).*cos(q3).*sin(q2).*sin( ...
  q4)).*sin(q6)).*sin(q7)).^2).^(-1)).*(1+(cos(q7).*(cos(q6).*(cos(q5).*(( ...
  -1).*cos(q3).*cos(q4).*sin(q2)+cos(q2).*sin(q4))+sin(q2).*sin(q3).*sin( ...
  q5))+((-1).*cos(q2).*cos(q4)+(-1).*cos(q3).*sin(q2).*sin(q4)).*sin(q6))+ ...
  (cos(q5).*sin(q2).*sin(q3)+(-1).*((-1).*cos(q3).*cos(q4).*sin(q2)+cos( ...
  q2).*sin(q4)).*sin(q5)).*sin(q7)).^2.*(((-1).*cos(q6).*((-1).*cos(q2).* ...
  cos(q4)+(-1).*cos(q3).*sin(q2).*sin(q4))+(cos(q5).*((-1).*cos(q3).*cos( ...
  q4).*sin(q2)+cos(q2).*sin(q4))+sin(q2).*sin(q3).*sin(q5)).*sin(q6)).^2+( ...
  cos(q7).*(cos(q5).*sin(q2).*sin(q3)+(-1).*((-1).*cos(q3).*cos(q4).*sin( ...
  q2)+cos(q2).*sin(q4)).*sin(q5))+(-1).*(cos(q6).*(cos(q5).*((-1).*cos(q3) ...
  .*cos(q4).*sin(q2)+cos(q2).*sin(q4))+sin(q2).*sin(q3).*sin(q5))+((-1).* ...
  cos(q2).*cos(q4)+(-1).*cos(q3).*sin(q2).*sin(q4)).*sin(q6)).*sin(q7)) ...
  .^2).^(-1)).^(-2).*((-1/2).*(cos(q7).*(cos(q6).*(cos(q5).*((-1).*cos(q3) ...
  .*cos(q4).*sin(q2)+cos(q2).*sin(q4))+sin(q2).*sin(q3).*sin(q5))+((-1).* ...
  cos(q2).*cos(q4)+(-1).*cos(q3).*sin(q2).*sin(q4)).*sin(q6))+(cos(q5).* ...
  sin(q2).*sin(q3)+(-1).*((-1).*cos(q3).*cos(q4).*sin(q2)+cos(q2).*sin(q4) ...
  ).*sin(q5)).*sin(q7)).*(2.*((-1).*cos(q6).*sin(q2).*sin(q3).*sin(q4)+( ...
  cos(q4).*cos(q5).*sin(q2).*sin(q3)+cos(q3).*sin(q2).*sin(q5)).*sin(q6)) ...
  .*((-1).*cos(q6).*((-1).*cos(q2).*cos(q4)+(-1).*cos(q3).*sin(q2).*sin( ...
  q4))+(cos(q5).*((-1).*cos(q3).*cos(q4).*sin(q2)+cos(q2).*sin(q4))+sin( ...
  q2).*sin(q3).*sin(q5)).*sin(q6))+2.*(cos(q7).*(cos(q3).*cos(q5).*sin(q2) ...
  +(-1).*cos(q4).*sin(q2).*sin(q3).*sin(q5))+(-1).*(cos(q6).*(cos(q4).* ...
  cos(q5).*sin(q2).*sin(q3)+cos(q3).*sin(q2).*sin(q5))+sin(q2).*sin(q3).* ...
  sin(q4).*sin(q6)).*sin(q7)).*(cos(q7).*(cos(q5).*sin(q2).*sin(q3)+(-1).* ...
  ((-1).*cos(q3).*cos(q4).*sin(q2)+cos(q2).*sin(q4)).*sin(q5))+(-1).*(cos( ...
  q6).*(cos(q5).*((-1).*cos(q3).*cos(q4).*sin(q2)+cos(q2).*sin(q4))+sin( ...
  q2).*sin(q3).*sin(q5))+((-1).*cos(q2).*cos(q4)+(-1).*cos(q3).*sin(q2).* ...
  sin(q4)).*sin(q6)).*sin(q7))).*(((-1).*cos(q6).*((-1).*cos(q2).*cos(q4)+ ...
  (-1).*cos(q3).*sin(q2).*sin(q4))+(cos(q5).*((-1).*cos(q3).*cos(q4).*sin( ...
  q2)+cos(q2).*sin(q4))+sin(q2).*sin(q3).*sin(q5)).*sin(q6)).^2+(cos(q7).* ...
  (cos(q5).*sin(q2).*sin(q3)+(-1).*((-1).*cos(q3).*cos(q4).*sin(q2)+cos( ...
  q2).*sin(q4)).*sin(q5))+(-1).*(cos(q6).*(cos(q5).*((-1).*cos(q3).*cos( ...
  q4).*sin(q2)+cos(q2).*sin(q4))+sin(q2).*sin(q3).*sin(q5))+((-1).*cos(q2) ...
  .*cos(q4)+(-1).*cos(q3).*sin(q2).*sin(q4)).*sin(q6)).*sin(q7)).^2).^( ...
  -3/2)+(cos(q7).*(cos(q6).*(cos(q4).*cos(q5).*sin(q2).*sin(q3)+cos(q3).* ...
  sin(q2).*sin(q5))+sin(q2).*sin(q3).*sin(q4).*sin(q6))+(cos(q3).*cos(q5) ...
  .*sin(q2)+(-1).*cos(q4).*sin(q2).*sin(q3).*sin(q5)).*sin(q7)).*(((-1).* ...
  cos(q6).*((-1).*cos(q2).*cos(q4)+(-1).*cos(q3).*sin(q2).*sin(q4))+(cos( ...
  q5).*((-1).*cos(q3).*cos(q4).*sin(q2)+cos(q2).*sin(q4))+sin(q2).*sin(q3) ...
  .*sin(q5)).*sin(q6)).^2+(cos(q7).*(cos(q5).*sin(q2).*sin(q3)+(-1).*((-1) ...
  .*cos(q3).*cos(q4).*sin(q2)+cos(q2).*sin(q4)).*sin(q5))+(-1).*(cos(q6).* ...
  (cos(q5).*((-1).*cos(q3).*cos(q4).*sin(q2)+cos(q2).*sin(q4))+sin(q2).* ...
  sin(q3).*sin(q5))+((-1).*cos(q2).*cos(q4)+(-1).*cos(q3).*sin(q2).*sin( ...
  q4)).*sin(q6)).*sin(q7)).^2).^(-1/2));

Jxe254 = (-1).*((-1).*(cos(q7).*(cos(q6).*( ...
  cos(q5).*((-1).*cos(q3).*cos(q4).*sin(q2)+cos(q2).*sin(q4))+sin(q2).* ...
  sin(q3).*sin(q5))+((-1).*cos(q2).*cos(q4)+(-1).*cos(q3).*sin(q2).*sin( ...
  q4)).*sin(q6))+(cos(q5).*sin(q2).*sin(q3)+(-1).*((-1).*cos(q3).*cos(q4) ...
  .*sin(q2)+cos(q2).*sin(q4)).*sin(q5)).*sin(q7)).^2.*(2.*((-1).*cos(q6).* ...
  ((-1).*cos(q3).*cos(q4).*sin(q2)+cos(q2).*sin(q4))+cos(q5).*(cos(q2).* ...
  cos(q4)+cos(q3).*sin(q2).*sin(q4)).*sin(q6)).*((-1).*cos(q6).*((-1).* ...
  cos(q2).*cos(q4)+(-1).*cos(q3).*sin(q2).*sin(q4))+(cos(q5).*((-1).*cos( ...
  q3).*cos(q4).*sin(q2)+cos(q2).*sin(q4))+sin(q2).*sin(q3).*sin(q5)).*sin( ...
  q6))+2.*((-1).*cos(q7).*(cos(q2).*cos(q4)+cos(q3).*sin(q2).*sin(q4)).* ...
  sin(q5)+(-1).*(cos(q5).*cos(q6).*(cos(q2).*cos(q4)+cos(q3).*sin(q2).* ...
  sin(q4))+((-1).*cos(q3).*cos(q4).*sin(q2)+cos(q2).*sin(q4)).*sin(q6)).* ...
  sin(q7)).*(cos(q7).*(cos(q5).*sin(q2).*sin(q3)+(-1).*((-1).*cos(q3).* ...
  cos(q4).*sin(q2)+cos(q2).*sin(q4)).*sin(q5))+(-1).*(cos(q6).*(cos(q5).*( ...
  (-1).*cos(q3).*cos(q4).*sin(q2)+cos(q2).*sin(q4))+sin(q2).*sin(q3).*sin( ...
  q5))+((-1).*cos(q2).*cos(q4)+(-1).*cos(q3).*sin(q2).*sin(q4)).*sin(q6)) ...
  .*sin(q7))).*(((-1).*cos(q6).*((-1).*cos(q2).*cos(q4)+(-1).*cos(q3).* ...
  sin(q2).*sin(q4))+(cos(q5).*((-1).*cos(q3).*cos(q4).*sin(q2)+cos(q2).* ...
  sin(q4))+sin(q2).*sin(q3).*sin(q5)).*sin(q6)).^2+(cos(q7).*(cos(q5).* ...
  sin(q2).*sin(q3)+(-1).*((-1).*cos(q3).*cos(q4).*sin(q2)+cos(q2).*sin(q4) ...
  ).*sin(q5))+(-1).*(cos(q6).*(cos(q5).*((-1).*cos(q3).*cos(q4).*sin(q2)+ ...
  cos(q2).*sin(q4))+sin(q2).*sin(q3).*sin(q5))+((-1).*cos(q2).*cos(q4)+( ...
  -1).*cos(q3).*sin(q2).*sin(q4)).*sin(q6)).*sin(q7)).^2).^(-2)+2.*(cos( ...
  q7).*(cos(q5).*cos(q6).*(cos(q2).*cos(q4)+cos(q3).*sin(q2).*sin(q4))+(( ...
  -1).*cos(q3).*cos(q4).*sin(q2)+cos(q2).*sin(q4)).*sin(q6))+(-1).*(cos( ...
  q2).*cos(q4)+cos(q3).*sin(q2).*sin(q4)).*sin(q5).*sin(q7)).*(cos(q7).*( ...
  cos(q6).*(cos(q5).*((-1).*cos(q3).*cos(q4).*sin(q2)+cos(q2).*sin(q4))+ ...
  sin(q2).*sin(q3).*sin(q5))+((-1).*cos(q2).*cos(q4)+(-1).*cos(q3).*sin( ...
  q2).*sin(q4)).*sin(q6))+(cos(q5).*sin(q2).*sin(q3)+(-1).*((-1).*cos(q3) ...
  .*cos(q4).*sin(q2)+cos(q2).*sin(q4)).*sin(q5)).*sin(q7)).*(((-1).*cos( ...
  q6).*((-1).*cos(q2).*cos(q4)+(-1).*cos(q3).*sin(q2).*sin(q4))+(cos(q5).* ...
  ((-1).*cos(q3).*cos(q4).*sin(q2)+cos(q2).*sin(q4))+sin(q2).*sin(q3).* ...
  sin(q5)).*sin(q6)).^2+(cos(q7).*(cos(q5).*sin(q2).*sin(q3)+(-1).*((-1).* ...
  cos(q3).*cos(q4).*sin(q2)+cos(q2).*sin(q4)).*sin(q5))+(-1).*(cos(q6).*( ...
  cos(q5).*((-1).*cos(q3).*cos(q4).*sin(q2)+cos(q2).*sin(q4))+sin(q2).* ...
  sin(q3).*sin(q5))+((-1).*cos(q2).*cos(q4)+(-1).*cos(q3).*sin(q2).*sin( ...
  q4)).*sin(q6)).*sin(q7)).^2).^(-1)).*(1+(cos(q7).*(cos(q6).*(cos(q5).*(( ...
  -1).*cos(q3).*cos(q4).*sin(q2)+cos(q2).*sin(q4))+sin(q2).*sin(q3).*sin( ...
  q5))+((-1).*cos(q2).*cos(q4)+(-1).*cos(q3).*sin(q2).*sin(q4)).*sin(q6))+ ...
  (cos(q5).*sin(q2).*sin(q3)+(-1).*((-1).*cos(q3).*cos(q4).*sin(q2)+cos( ...
  q2).*sin(q4)).*sin(q5)).*sin(q7)).^2.*(((-1).*cos(q6).*((-1).*cos(q2).* ...
  cos(q4)+(-1).*cos(q3).*sin(q2).*sin(q4))+(cos(q5).*((-1).*cos(q3).*cos( ...
  q4).*sin(q2)+cos(q2).*sin(q4))+sin(q2).*sin(q3).*sin(q5)).*sin(q6)).^2+( ...
  cos(q7).*(cos(q5).*sin(q2).*sin(q3)+(-1).*((-1).*cos(q3).*cos(q4).*sin( ...
  q2)+cos(q2).*sin(q4)).*sin(q5))+(-1).*(cos(q6).*(cos(q5).*((-1).*cos(q3) ...
  .*cos(q4).*sin(q2)+cos(q2).*sin(q4))+sin(q2).*sin(q3).*sin(q5))+((-1).* ...
  cos(q2).*cos(q4)+(-1).*cos(q3).*sin(q2).*sin(q4)).*sin(q6)).*sin(q7)) ...
  .^2).^(-1)).^(-2).*((-1/2).*(cos(q7).*(cos(q6).*(cos(q5).*((-1).*cos(q3) ...
  .*cos(q4).*sin(q2)+cos(q2).*sin(q4))+sin(q2).*sin(q3).*sin(q5))+((-1).* ...
  cos(q2).*cos(q4)+(-1).*cos(q3).*sin(q2).*sin(q4)).*sin(q6))+(cos(q5).* ...
  sin(q2).*sin(q3)+(-1).*((-1).*cos(q3).*cos(q4).*sin(q2)+cos(q2).*sin(q4) ...
  ).*sin(q5)).*sin(q7)).*(2.*((-1).*cos(q6).*((-1).*cos(q3).*cos(q4).*sin( ...
  q2)+cos(q2).*sin(q4))+cos(q5).*(cos(q2).*cos(q4)+cos(q3).*sin(q2).*sin( ...
  q4)).*sin(q6)).*((-1).*cos(q6).*((-1).*cos(q2).*cos(q4)+(-1).*cos(q3).* ...
  sin(q2).*sin(q4))+(cos(q5).*((-1).*cos(q3).*cos(q4).*sin(q2)+cos(q2).* ...
  sin(q4))+sin(q2).*sin(q3).*sin(q5)).*sin(q6))+2.*((-1).*cos(q7).*(cos( ...
  q2).*cos(q4)+cos(q3).*sin(q2).*sin(q4)).*sin(q5)+(-1).*(cos(q5).*cos(q6) ...
  .*(cos(q2).*cos(q4)+cos(q3).*sin(q2).*sin(q4))+((-1).*cos(q3).*cos(q4).* ...
  sin(q2)+cos(q2).*sin(q4)).*sin(q6)).*sin(q7)).*(cos(q7).*(cos(q5).*sin( ...
  q2).*sin(q3)+(-1).*((-1).*cos(q3).*cos(q4).*sin(q2)+cos(q2).*sin(q4)).* ...
  sin(q5))+(-1).*(cos(q6).*(cos(q5).*((-1).*cos(q3).*cos(q4).*sin(q2)+cos( ...
  q2).*sin(q4))+sin(q2).*sin(q3).*sin(q5))+((-1).*cos(q2).*cos(q4)+(-1).* ...
  cos(q3).*sin(q2).*sin(q4)).*sin(q6)).*sin(q7))).*(((-1).*cos(q6).*((-1) ...
  .*cos(q2).*cos(q4)+(-1).*cos(q3).*sin(q2).*sin(q4))+(cos(q5).*((-1).* ...
  cos(q3).*cos(q4).*sin(q2)+cos(q2).*sin(q4))+sin(q2).*sin(q3).*sin(q5)).* ...
  sin(q6)).^2+(cos(q7).*(cos(q5).*sin(q2).*sin(q3)+(-1).*((-1).*cos(q3).* ...
  cos(q4).*sin(q2)+cos(q2).*sin(q4)).*sin(q5))+(-1).*(cos(q6).*(cos(q5).*( ...
  (-1).*cos(q3).*cos(q4).*sin(q2)+cos(q2).*sin(q4))+sin(q2).*sin(q3).*sin( ...
  q5))+((-1).*cos(q2).*cos(q4)+(-1).*cos(q3).*sin(q2).*sin(q4)).*sin(q6)) ...
  .*sin(q7)).^2).^(-3/2)+(cos(q7).*(cos(q5).*cos(q6).*(cos(q2).*cos(q4)+ ...
  cos(q3).*sin(q2).*sin(q4))+((-1).*cos(q3).*cos(q4).*sin(q2)+cos(q2).* ...
  sin(q4)).*sin(q6))+(-1).*(cos(q2).*cos(q4)+cos(q3).*sin(q2).*sin(q4)).* ...
  sin(q5).*sin(q7)).*(((-1).*cos(q6).*((-1).*cos(q2).*cos(q4)+(-1).*cos( ...
  q3).*sin(q2).*sin(q4))+(cos(q5).*((-1).*cos(q3).*cos(q4).*sin(q2)+cos( ...
  q2).*sin(q4))+sin(q2).*sin(q3).*sin(q5)).*sin(q6)).^2+(cos(q7).*(cos(q5) ...
  .*sin(q2).*sin(q3)+(-1).*((-1).*cos(q3).*cos(q4).*sin(q2)+cos(q2).*sin( ...
  q4)).*sin(q5))+(-1).*(cos(q6).*(cos(q5).*((-1).*cos(q3).*cos(q4).*sin( ...
  q2)+cos(q2).*sin(q4))+sin(q2).*sin(q3).*sin(q5))+((-1).*cos(q2).*cos(q4) ...
  +(-1).*cos(q3).*sin(q2).*sin(q4)).*sin(q6)).*sin(q7)).^2).^(-1/2))+(1+( ...
  cos(q7).*(cos(q6).*(cos(q5).*((-1).*cos(q3).*cos(q4).*sin(q2)+cos(q2).* ...
  sin(q4))+sin(q2).*sin(q3).*sin(q5))+((-1).*cos(q2).*cos(q4)+(-1).*cos( ...
  q3).*sin(q2).*sin(q4)).*sin(q6))+(cos(q5).*sin(q2).*sin(q3)+(-1).*((-1) ...
  .*cos(q3).*cos(q4).*sin(q2)+cos(q2).*sin(q4)).*sin(q5)).*sin(q7)).^2.*(( ...
  (-1).*cos(q6).*((-1).*cos(q2).*cos(q4)+(-1).*cos(q3).*sin(q2).*sin(q4))+ ...
  (cos(q5).*((-1).*cos(q3).*cos(q4).*sin(q2)+cos(q2).*sin(q4))+sin(q2).* ...
  sin(q3).*sin(q5)).*sin(q6)).^2+(cos(q7).*(cos(q5).*sin(q2).*sin(q3)+(-1) ...
  .*((-1).*cos(q3).*cos(q4).*sin(q2)+cos(q2).*sin(q4)).*sin(q5))+(-1).*( ...
  cos(q6).*(cos(q5).*((-1).*cos(q3).*cos(q4).*sin(q2)+cos(q2).*sin(q4))+ ...
  sin(q2).*sin(q3).*sin(q5))+((-1).*cos(q2).*cos(q4)+(-1).*cos(q3).*sin( ...
  q2).*sin(q4)).*sin(q6)).*sin(q7)).^2).^(-1)).^(-1).*((3/4).*(cos(q7).*( ...
  cos(q6).*(cos(q5).*((-1).*cos(q3).*cos(q4).*sin(q2)+cos(q2).*sin(q4))+ ...
  sin(q2).*sin(q3).*sin(q5))+((-1).*cos(q2).*cos(q4)+(-1).*cos(q3).*sin( ...
  q2).*sin(q4)).*sin(q6))+(cos(q5).*sin(q2).*sin(q3)+(-1).*((-1).*cos(q3) ...
  .*cos(q4).*sin(q2)+cos(q2).*sin(q4)).*sin(q5)).*sin(q7)).*(2.*((-1).* ...
  cos(q6).*((-1).*cos(q3).*cos(q4).*sin(q2)+cos(q2).*sin(q4))+cos(q5).*( ...
  cos(q2).*cos(q4)+cos(q3).*sin(q2).*sin(q4)).*sin(q6)).*((-1).*cos(q6).*( ...
  (-1).*cos(q2).*cos(q4)+(-1).*cos(q3).*sin(q2).*sin(q4))+(cos(q5).*((-1) ...
  .*cos(q3).*cos(q4).*sin(q2)+cos(q2).*sin(q4))+sin(q2).*sin(q3).*sin(q5)) ...
  .*sin(q6))+2.*((-1).*cos(q7).*(cos(q2).*cos(q4)+cos(q3).*sin(q2).*sin( ...
  q4)).*sin(q5)+(-1).*(cos(q5).*cos(q6).*(cos(q2).*cos(q4)+cos(q3).*sin( ...
  q2).*sin(q4))+((-1).*cos(q3).*cos(q4).*sin(q2)+cos(q2).*sin(q4)).*sin( ...
  q6)).*sin(q7)).*(cos(q7).*(cos(q5).*sin(q2).*sin(q3)+(-1).*((-1).*cos( ...
  q3).*cos(q4).*sin(q2)+cos(q2).*sin(q4)).*sin(q5))+(-1).*(cos(q6).*(cos( ...
  q5).*((-1).*cos(q3).*cos(q4).*sin(q2)+cos(q2).*sin(q4))+sin(q2).*sin(q3) ...
  .*sin(q5))+((-1).*cos(q2).*cos(q4)+(-1).*cos(q3).*sin(q2).*sin(q4)).* ...
  sin(q6)).*sin(q7))).^2.*(((-1).*cos(q6).*((-1).*cos(q2).*cos(q4)+(-1).* ...
  cos(q3).*sin(q2).*sin(q4))+(cos(q5).*((-1).*cos(q3).*cos(q4).*sin(q2)+ ...
  cos(q2).*sin(q4))+sin(q2).*sin(q3).*sin(q5)).*sin(q6)).^2+(cos(q7).*( ...
  cos(q5).*sin(q2).*sin(q3)+(-1).*((-1).*cos(q3).*cos(q4).*sin(q2)+cos(q2) ...
  .*sin(q4)).*sin(q5))+(-1).*(cos(q6).*(cos(q5).*((-1).*cos(q3).*cos(q4).* ...
  sin(q2)+cos(q2).*sin(q4))+sin(q2).*sin(q3).*sin(q5))+((-1).*cos(q2).* ...
  cos(q4)+(-1).*cos(q3).*sin(q2).*sin(q4)).*sin(q6)).*sin(q7)).^2).^(-5/2) ...
  +(-1).*(cos(q7).*(cos(q5).*cos(q6).*(cos(q2).*cos(q4)+cos(q3).*sin(q2).* ...
  sin(q4))+((-1).*cos(q3).*cos(q4).*sin(q2)+cos(q2).*sin(q4)).*sin(q6))+( ...
  -1).*(cos(q2).*cos(q4)+cos(q3).*sin(q2).*sin(q4)).*sin(q5).*sin(q7)).*( ...
  2.*((-1).*cos(q6).*((-1).*cos(q3).*cos(q4).*sin(q2)+cos(q2).*sin(q4))+ ...
  cos(q5).*(cos(q2).*cos(q4)+cos(q3).*sin(q2).*sin(q4)).*sin(q6)).*((-1).* ...
  cos(q6).*((-1).*cos(q2).*cos(q4)+(-1).*cos(q3).*sin(q2).*sin(q4))+(cos( ...
  q5).*((-1).*cos(q3).*cos(q4).*sin(q2)+cos(q2).*sin(q4))+sin(q2).*sin(q3) ...
  .*sin(q5)).*sin(q6))+2.*((-1).*cos(q7).*(cos(q2).*cos(q4)+cos(q3).*sin( ...
  q2).*sin(q4)).*sin(q5)+(-1).*(cos(q5).*cos(q6).*(cos(q2).*cos(q4)+cos( ...
  q3).*sin(q2).*sin(q4))+((-1).*cos(q3).*cos(q4).*sin(q2)+cos(q2).*sin(q4) ...
  ).*sin(q6)).*sin(q7)).*(cos(q7).*(cos(q5).*sin(q2).*sin(q3)+(-1).*((-1) ...
  .*cos(q3).*cos(q4).*sin(q2)+cos(q2).*sin(q4)).*sin(q5))+(-1).*(cos(q6).* ...
  (cos(q5).*((-1).*cos(q3).*cos(q4).*sin(q2)+cos(q2).*sin(q4))+sin(q2).* ...
  sin(q3).*sin(q5))+((-1).*cos(q2).*cos(q4)+(-1).*cos(q3).*sin(q2).*sin( ...
  q4)).*sin(q6)).*sin(q7))).*(((-1).*cos(q6).*((-1).*cos(q2).*cos(q4)+(-1) ...
  .*cos(q3).*sin(q2).*sin(q4))+(cos(q5).*((-1).*cos(q3).*cos(q4).*sin(q2)+ ...
  cos(q2).*sin(q4))+sin(q2).*sin(q3).*sin(q5)).*sin(q6)).^2+(cos(q7).*( ...
  cos(q5).*sin(q2).*sin(q3)+(-1).*((-1).*cos(q3).*cos(q4).*sin(q2)+cos(q2) ...
  .*sin(q4)).*sin(q5))+(-1).*(cos(q6).*(cos(q5).*((-1).*cos(q3).*cos(q4).* ...
  sin(q2)+cos(q2).*sin(q4))+sin(q2).*sin(q3).*sin(q5))+((-1).*cos(q2).* ...
  cos(q4)+(-1).*cos(q3).*sin(q2).*sin(q4)).*sin(q6)).*sin(q7)).^2).^(-3/2) ...
  +(cos(q7).*(cos(q5).*cos(q6).*(cos(q3).*cos(q4).*sin(q2)+(-1).*cos(q2).* ...
  sin(q4))+(cos(q2).*cos(q4)+cos(q3).*sin(q2).*sin(q4)).*sin(q6))+(-1).*( ...
  cos(q3).*cos(q4).*sin(q2)+(-1).*cos(q2).*sin(q4)).*sin(q5).*sin(q7)).*(( ...
  (-1).*cos(q6).*((-1).*cos(q2).*cos(q4)+(-1).*cos(q3).*sin(q2).*sin(q4))+ ...
  (cos(q5).*((-1).*cos(q3).*cos(q4).*sin(q2)+cos(q2).*sin(q4))+sin(q2).* ...
  sin(q3).*sin(q5)).*sin(q6)).^2+(cos(q7).*(cos(q5).*sin(q2).*sin(q3)+(-1) ...
  .*((-1).*cos(q3).*cos(q4).*sin(q2)+cos(q2).*sin(q4)).*sin(q5))+(-1).*( ...
  cos(q6).*(cos(q5).*((-1).*cos(q3).*cos(q4).*sin(q2)+cos(q2).*sin(q4))+ ...
  sin(q2).*sin(q3).*sin(q5))+((-1).*cos(q2).*cos(q4)+(-1).*cos(q3).*sin( ...
  q2).*sin(q4)).*sin(q6)).*sin(q7)).^2).^(-1/2)+(-1/2).*(cos(q7).*(cos(q6) ...
  .*(cos(q5).*((-1).*cos(q3).*cos(q4).*sin(q2)+cos(q2).*sin(q4))+sin(q2).* ...
  sin(q3).*sin(q5))+((-1).*cos(q2).*cos(q4)+(-1).*cos(q3).*sin(q2).*sin( ...
  q4)).*sin(q6))+(cos(q5).*sin(q2).*sin(q3)+(-1).*((-1).*cos(q3).*cos(q4) ...
  .*sin(q2)+cos(q2).*sin(q4)).*sin(q5)).*sin(q7)).*(((-1).*cos(q6).*((-1) ...
  .*cos(q2).*cos(q4)+(-1).*cos(q3).*sin(q2).*sin(q4))+(cos(q5).*((-1).* ...
  cos(q3).*cos(q4).*sin(q2)+cos(q2).*sin(q4))+sin(q2).*sin(q3).*sin(q5)).* ...
  sin(q6)).^2+(cos(q7).*(cos(q5).*sin(q2).*sin(q3)+(-1).*((-1).*cos(q3).* ...
  cos(q4).*sin(q2)+cos(q2).*sin(q4)).*sin(q5))+(-1).*(cos(q6).*(cos(q5).*( ...
  (-1).*cos(q3).*cos(q4).*sin(q2)+cos(q2).*sin(q4))+sin(q2).*sin(q3).*sin( ...
  q5))+((-1).*cos(q2).*cos(q4)+(-1).*cos(q3).*sin(q2).*sin(q4)).*sin(q6)) ...
  .*sin(q7)).^2).^(-3/2).*(2.*((-1).*cos(q6).*((-1).*cos(q3).*cos(q4).* ...
  sin(q2)+cos(q2).*sin(q4))+cos(q5).*(cos(q2).*cos(q4)+cos(q3).*sin(q2).* ...
  sin(q4)).*sin(q6)).^2+2.*((-1).*cos(q6).*(cos(q2).*cos(q4)+cos(q3).*sin( ...
  q2).*sin(q4))+cos(q5).*(cos(q3).*cos(q4).*sin(q2)+(-1).*cos(q2).*sin(q4) ...
  ).*sin(q6)).*((-1).*cos(q6).*((-1).*cos(q2).*cos(q4)+(-1).*cos(q3).*sin( ...
  q2).*sin(q4))+(cos(q5).*((-1).*cos(q3).*cos(q4).*sin(q2)+cos(q2).*sin( ...
  q4))+sin(q2).*sin(q3).*sin(q5)).*sin(q6))+2.*((-1).*cos(q7).*(cos(q2).* ...
  cos(q4)+cos(q3).*sin(q2).*sin(q4)).*sin(q5)+(-1).*(cos(q5).*cos(q6).*( ...
  cos(q2).*cos(q4)+cos(q3).*sin(q2).*sin(q4))+((-1).*cos(q3).*cos(q4).* ...
  sin(q2)+cos(q2).*sin(q4)).*sin(q6)).*sin(q7)).^2+2.*(cos(q7).*(cos(q5).* ...
  sin(q2).*sin(q3)+(-1).*((-1).*cos(q3).*cos(q4).*sin(q2)+cos(q2).*sin(q4) ...
  ).*sin(q5))+(-1).*(cos(q6).*(cos(q5).*((-1).*cos(q3).*cos(q4).*sin(q2)+ ...
  cos(q2).*sin(q4))+sin(q2).*sin(q3).*sin(q5))+((-1).*cos(q2).*cos(q4)+( ...
  -1).*cos(q3).*sin(q2).*sin(q4)).*sin(q6)).*sin(q7)).*((-1).*cos(q7).*( ...
  cos(q3).*cos(q4).*sin(q2)+(-1).*cos(q2).*sin(q4)).*sin(q5)+(-1).*(cos( ...
  q5).*cos(q6).*(cos(q3).*cos(q4).*sin(q2)+(-1).*cos(q2).*sin(q4))+(cos( ...
  q2).*cos(q4)+cos(q3).*sin(q2).*sin(q4)).*sin(q6)).*sin(q7))));

Jxe255 = (-1).*(( ...
  -1).*(cos(q7).*(cos(q6).*(cos(q5).*((-1).*cos(q3).*cos(q4).*sin(q2)+cos( ...
  q2).*sin(q4))+sin(q2).*sin(q3).*sin(q5))+((-1).*cos(q2).*cos(q4)+(-1).* ...
  cos(q3).*sin(q2).*sin(q4)).*sin(q6))+(cos(q5).*sin(q2).*sin(q3)+(-1).*(( ...
  -1).*cos(q3).*cos(q4).*sin(q2)+cos(q2).*sin(q4)).*sin(q5)).*sin(q7)) ...
  .^2.*(2.*(cos(q5).*sin(q2).*sin(q3)+(-1).*((-1).*cos(q3).*cos(q4).*sin( ...
  q2)+cos(q2).*sin(q4)).*sin(q5)).*sin(q6).*((-1).*cos(q6).*((-1).*cos(q2) ...
  .*cos(q4)+(-1).*cos(q3).*sin(q2).*sin(q4))+(cos(q5).*((-1).*cos(q3).* ...
  cos(q4).*sin(q2)+cos(q2).*sin(q4))+sin(q2).*sin(q3).*sin(q5)).*sin(q6))+ ...
  2.*(cos(q7).*((-1).*cos(q5).*((-1).*cos(q3).*cos(q4).*sin(q2)+cos(q2).* ...
  sin(q4))+(-1).*sin(q2).*sin(q3).*sin(q5))+(-1).*cos(q6).*(cos(q5).*sin( ...
  q2).*sin(q3)+(-1).*((-1).*cos(q3).*cos(q4).*sin(q2)+cos(q2).*sin(q4)).* ...
  sin(q5)).*sin(q7)).*(cos(q7).*(cos(q5).*sin(q2).*sin(q3)+(-1).*((-1).* ...
  cos(q3).*cos(q4).*sin(q2)+cos(q2).*sin(q4)).*sin(q5))+(-1).*(cos(q6).*( ...
  cos(q5).*((-1).*cos(q3).*cos(q4).*sin(q2)+cos(q2).*sin(q4))+sin(q2).* ...
  sin(q3).*sin(q5))+((-1).*cos(q2).*cos(q4)+(-1).*cos(q3).*sin(q2).*sin( ...
  q4)).*sin(q6)).*sin(q7))).*(((-1).*cos(q6).*((-1).*cos(q2).*cos(q4)+(-1) ...
  .*cos(q3).*sin(q2).*sin(q4))+(cos(q5).*((-1).*cos(q3).*cos(q4).*sin(q2)+ ...
  cos(q2).*sin(q4))+sin(q2).*sin(q3).*sin(q5)).*sin(q6)).^2+(cos(q7).*( ...
  cos(q5).*sin(q2).*sin(q3)+(-1).*((-1).*cos(q3).*cos(q4).*sin(q2)+cos(q2) ...
  .*sin(q4)).*sin(q5))+(-1).*(cos(q6).*(cos(q5).*((-1).*cos(q3).*cos(q4).* ...
  sin(q2)+cos(q2).*sin(q4))+sin(q2).*sin(q3).*sin(q5))+((-1).*cos(q2).* ...
  cos(q4)+(-1).*cos(q3).*sin(q2).*sin(q4)).*sin(q6)).*sin(q7)).^2).^(-2)+ ...
  2.*(cos(q6).*cos(q7).*(cos(q5).*sin(q2).*sin(q3)+(-1).*((-1).*cos(q3).* ...
  cos(q4).*sin(q2)+cos(q2).*sin(q4)).*sin(q5))+((-1).*cos(q5).*((-1).*cos( ...
  q3).*cos(q4).*sin(q2)+cos(q2).*sin(q4))+(-1).*sin(q2).*sin(q3).*sin(q5)) ...
  .*sin(q7)).*(cos(q7).*(cos(q6).*(cos(q5).*((-1).*cos(q3).*cos(q4).*sin( ...
  q2)+cos(q2).*sin(q4))+sin(q2).*sin(q3).*sin(q5))+((-1).*cos(q2).*cos(q4) ...
  +(-1).*cos(q3).*sin(q2).*sin(q4)).*sin(q6))+(cos(q5).*sin(q2).*sin(q3)+( ...
  -1).*((-1).*cos(q3).*cos(q4).*sin(q2)+cos(q2).*sin(q4)).*sin(q5)).*sin( ...
  q7)).*(((-1).*cos(q6).*((-1).*cos(q2).*cos(q4)+(-1).*cos(q3).*sin(q2).* ...
  sin(q4))+(cos(q5).*((-1).*cos(q3).*cos(q4).*sin(q2)+cos(q2).*sin(q4))+ ...
  sin(q2).*sin(q3).*sin(q5)).*sin(q6)).^2+(cos(q7).*(cos(q5).*sin(q2).* ...
  sin(q3)+(-1).*((-1).*cos(q3).*cos(q4).*sin(q2)+cos(q2).*sin(q4)).*sin( ...
  q5))+(-1).*(cos(q6).*(cos(q5).*((-1).*cos(q3).*cos(q4).*sin(q2)+cos(q2) ...
  .*sin(q4))+sin(q2).*sin(q3).*sin(q5))+((-1).*cos(q2).*cos(q4)+(-1).*cos( ...
  q3).*sin(q2).*sin(q4)).*sin(q6)).*sin(q7)).^2).^(-1)).*(1+(cos(q7).*( ...
  cos(q6).*(cos(q5).*((-1).*cos(q3).*cos(q4).*sin(q2)+cos(q2).*sin(q4))+ ...
  sin(q2).*sin(q3).*sin(q5))+((-1).*cos(q2).*cos(q4)+(-1).*cos(q3).*sin( ...
  q2).*sin(q4)).*sin(q6))+(cos(q5).*sin(q2).*sin(q3)+(-1).*((-1).*cos(q3) ...
  .*cos(q4).*sin(q2)+cos(q2).*sin(q4)).*sin(q5)).*sin(q7)).^2.*(((-1).* ...
  cos(q6).*((-1).*cos(q2).*cos(q4)+(-1).*cos(q3).*sin(q2).*sin(q4))+(cos( ...
  q5).*((-1).*cos(q3).*cos(q4).*sin(q2)+cos(q2).*sin(q4))+sin(q2).*sin(q3) ...
  .*sin(q5)).*sin(q6)).^2+(cos(q7).*(cos(q5).*sin(q2).*sin(q3)+(-1).*((-1) ...
  .*cos(q3).*cos(q4).*sin(q2)+cos(q2).*sin(q4)).*sin(q5))+(-1).*(cos(q6).* ...
  (cos(q5).*((-1).*cos(q3).*cos(q4).*sin(q2)+cos(q2).*sin(q4))+sin(q2).* ...
  sin(q3).*sin(q5))+((-1).*cos(q2).*cos(q4)+(-1).*cos(q3).*sin(q2).*sin( ...
  q4)).*sin(q6)).*sin(q7)).^2).^(-1)).^(-2).*((-1/2).*(cos(q7).*(cos(q6).* ...
  (cos(q5).*((-1).*cos(q3).*cos(q4).*sin(q2)+cos(q2).*sin(q4))+sin(q2).* ...
  sin(q3).*sin(q5))+((-1).*cos(q2).*cos(q4)+(-1).*cos(q3).*sin(q2).*sin( ...
  q4)).*sin(q6))+(cos(q5).*sin(q2).*sin(q3)+(-1).*((-1).*cos(q3).*cos(q4) ...
  .*sin(q2)+cos(q2).*sin(q4)).*sin(q5)).*sin(q7)).*(2.*(cos(q5).*sin(q2).* ...
  sin(q3)+(-1).*((-1).*cos(q3).*cos(q4).*sin(q2)+cos(q2).*sin(q4)).*sin( ...
  q5)).*sin(q6).*((-1).*cos(q6).*((-1).*cos(q2).*cos(q4)+(-1).*cos(q3).* ...
  sin(q2).*sin(q4))+(cos(q5).*((-1).*cos(q3).*cos(q4).*sin(q2)+cos(q2).* ...
  sin(q4))+sin(q2).*sin(q3).*sin(q5)).*sin(q6))+2.*(cos(q7).*((-1).*cos( ...
  q5).*((-1).*cos(q3).*cos(q4).*sin(q2)+cos(q2).*sin(q4))+(-1).*sin(q2).* ...
  sin(q3).*sin(q5))+(-1).*cos(q6).*(cos(q5).*sin(q2).*sin(q3)+(-1).*((-1) ...
  .*cos(q3).*cos(q4).*sin(q2)+cos(q2).*sin(q4)).*sin(q5)).*sin(q7)).*(cos( ...
  q7).*(cos(q5).*sin(q2).*sin(q3)+(-1).*((-1).*cos(q3).*cos(q4).*sin(q2)+ ...
  cos(q2).*sin(q4)).*sin(q5))+(-1).*(cos(q6).*(cos(q5).*((-1).*cos(q3).* ...
  cos(q4).*sin(q2)+cos(q2).*sin(q4))+sin(q2).*sin(q3).*sin(q5))+((-1).* ...
  cos(q2).*cos(q4)+(-1).*cos(q3).*sin(q2).*sin(q4)).*sin(q6)).*sin(q7))).* ...
  (((-1).*cos(q6).*((-1).*cos(q2).*cos(q4)+(-1).*cos(q3).*sin(q2).*sin(q4) ...
  )+(cos(q5).*((-1).*cos(q3).*cos(q4).*sin(q2)+cos(q2).*sin(q4))+sin(q2).* ...
  sin(q3).*sin(q5)).*sin(q6)).^2+(cos(q7).*(cos(q5).*sin(q2).*sin(q3)+(-1) ...
  .*((-1).*cos(q3).*cos(q4).*sin(q2)+cos(q2).*sin(q4)).*sin(q5))+(-1).*( ...
  cos(q6).*(cos(q5).*((-1).*cos(q3).*cos(q4).*sin(q2)+cos(q2).*sin(q4))+ ...
  sin(q2).*sin(q3).*sin(q5))+((-1).*cos(q2).*cos(q4)+(-1).*cos(q3).*sin( ...
  q2).*sin(q4)).*sin(q6)).*sin(q7)).^2).^(-3/2)+(cos(q6).*cos(q7).*(cos( ...
  q5).*sin(q2).*sin(q3)+(-1).*((-1).*cos(q3).*cos(q4).*sin(q2)+cos(q2).* ...
  sin(q4)).*sin(q5))+((-1).*cos(q5).*((-1).*cos(q3).*cos(q4).*sin(q2)+cos( ...
  q2).*sin(q4))+(-1).*sin(q2).*sin(q3).*sin(q5)).*sin(q7)).*(((-1).*cos( ...
  q6).*((-1).*cos(q2).*cos(q4)+(-1).*cos(q3).*sin(q2).*sin(q4))+(cos(q5).* ...
  ((-1).*cos(q3).*cos(q4).*sin(q2)+cos(q2).*sin(q4))+sin(q2).*sin(q3).* ...
  sin(q5)).*sin(q6)).^2+(cos(q7).*(cos(q5).*sin(q2).*sin(q3)+(-1).*((-1).* ...
  cos(q3).*cos(q4).*sin(q2)+cos(q2).*sin(q4)).*sin(q5))+(-1).*(cos(q6).*( ...
  cos(q5).*((-1).*cos(q3).*cos(q4).*sin(q2)+cos(q2).*sin(q4))+sin(q2).* ...
  sin(q3).*sin(q5))+((-1).*cos(q2).*cos(q4)+(-1).*cos(q3).*sin(q2).*sin( ...
  q4)).*sin(q6)).*sin(q7)).^2).^(-1/2))+(1+(cos(q7).*(cos(q6).*(cos(q5).*( ...
  (-1).*cos(q3).*cos(q4).*sin(q2)+cos(q2).*sin(q4))+sin(q2).*sin(q3).*sin( ...
  q5))+((-1).*cos(q2).*cos(q4)+(-1).*cos(q3).*sin(q2).*sin(q4)).*sin(q6))+ ...
  (cos(q5).*sin(q2).*sin(q3)+(-1).*((-1).*cos(q3).*cos(q4).*sin(q2)+cos( ...
  q2).*sin(q4)).*sin(q5)).*sin(q7)).^2.*(((-1).*cos(q6).*((-1).*cos(q2).* ...
  cos(q4)+(-1).*cos(q3).*sin(q2).*sin(q4))+(cos(q5).*((-1).*cos(q3).*cos( ...
  q4).*sin(q2)+cos(q2).*sin(q4))+sin(q2).*sin(q3).*sin(q5)).*sin(q6)).^2+( ...
  cos(q7).*(cos(q5).*sin(q2).*sin(q3)+(-1).*((-1).*cos(q3).*cos(q4).*sin( ...
  q2)+cos(q2).*sin(q4)).*sin(q5))+(-1).*(cos(q6).*(cos(q5).*((-1).*cos(q3) ...
  .*cos(q4).*sin(q2)+cos(q2).*sin(q4))+sin(q2).*sin(q3).*sin(q5))+((-1).* ...
  cos(q2).*cos(q4)+(-1).*cos(q3).*sin(q2).*sin(q4)).*sin(q6)).*sin(q7)) ...
  .^2).^(-1)).^(-1).*((3/4).*(cos(q7).*(cos(q6).*(cos(q5).*((-1).*cos(q3) ...
  .*cos(q4).*sin(q2)+cos(q2).*sin(q4))+sin(q2).*sin(q3).*sin(q5))+((-1).* ...
  cos(q2).*cos(q4)+(-1).*cos(q3).*sin(q2).*sin(q4)).*sin(q6))+(cos(q5).* ...
  sin(q2).*sin(q3)+(-1).*((-1).*cos(q3).*cos(q4).*sin(q2)+cos(q2).*sin(q4) ...
  ).*sin(q5)).*sin(q7)).*(2.*(cos(q5).*sin(q2).*sin(q3)+(-1).*((-1).*cos( ...
  q3).*cos(q4).*sin(q2)+cos(q2).*sin(q4)).*sin(q5)).*sin(q6).*((-1).*cos( ...
  q6).*((-1).*cos(q2).*cos(q4)+(-1).*cos(q3).*sin(q2).*sin(q4))+(cos(q5).* ...
  ((-1).*cos(q3).*cos(q4).*sin(q2)+cos(q2).*sin(q4))+sin(q2).*sin(q3).* ...
  sin(q5)).*sin(q6))+2.*(cos(q7).*((-1).*cos(q5).*((-1).*cos(q3).*cos(q4) ...
  .*sin(q2)+cos(q2).*sin(q4))+(-1).*sin(q2).*sin(q3).*sin(q5))+(-1).*cos( ...
  q6).*(cos(q5).*sin(q2).*sin(q3)+(-1).*((-1).*cos(q3).*cos(q4).*sin(q2)+ ...
  cos(q2).*sin(q4)).*sin(q5)).*sin(q7)).*(cos(q7).*(cos(q5).*sin(q2).*sin( ...
  q3)+(-1).*((-1).*cos(q3).*cos(q4).*sin(q2)+cos(q2).*sin(q4)).*sin(q5))+( ...
  -1).*(cos(q6).*(cos(q5).*((-1).*cos(q3).*cos(q4).*sin(q2)+cos(q2).*sin( ...
  q4))+sin(q2).*sin(q3).*sin(q5))+((-1).*cos(q2).*cos(q4)+(-1).*cos(q3).* ...
  sin(q2).*sin(q4)).*sin(q6)).*sin(q7))).^2.*(((-1).*cos(q6).*((-1).*cos( ...
  q2).*cos(q4)+(-1).*cos(q3).*sin(q2).*sin(q4))+(cos(q5).*((-1).*cos(q3).* ...
  cos(q4).*sin(q2)+cos(q2).*sin(q4))+sin(q2).*sin(q3).*sin(q5)).*sin(q6)) ...
  .^2+(cos(q7).*(cos(q5).*sin(q2).*sin(q3)+(-1).*((-1).*cos(q3).*cos(q4).* ...
  sin(q2)+cos(q2).*sin(q4)).*sin(q5))+(-1).*(cos(q6).*(cos(q5).*((-1).* ...
  cos(q3).*cos(q4).*sin(q2)+cos(q2).*sin(q4))+sin(q2).*sin(q3).*sin(q5))+( ...
  (-1).*cos(q2).*cos(q4)+(-1).*cos(q3).*sin(q2).*sin(q4)).*sin(q6)).*sin( ...
  q7)).^2).^(-5/2)+(-1/2).*(cos(q7).*(cos(q6).*(cos(q5).*((-1).*cos(q3).* ...
  cos(q4).*sin(q2)+cos(q2).*sin(q4))+sin(q2).*sin(q3).*sin(q5))+((-1).* ...
  cos(q2).*cos(q4)+(-1).*cos(q3).*sin(q2).*sin(q4)).*sin(q6))+(cos(q5).* ...
  sin(q2).*sin(q3)+(-1).*((-1).*cos(q3).*cos(q4).*sin(q2)+cos(q2).*sin(q4) ...
  ).*sin(q5)).*sin(q7)).*(2.*(cos(q5).*sin(q2).*sin(q3)+(-1).*((-1).*cos( ...
  q3).*cos(q4).*sin(q2)+cos(q2).*sin(q4)).*sin(q5)).^2.*sin(q6).^2+2.*(( ...
  -1).*cos(q5).*((-1).*cos(q3).*cos(q4).*sin(q2)+cos(q2).*sin(q4))+(-1).* ...
  sin(q2).*sin(q3).*sin(q5)).*sin(q6).*((-1).*cos(q6).*((-1).*cos(q2).* ...
  cos(q4)+(-1).*cos(q3).*sin(q2).*sin(q4))+(cos(q5).*((-1).*cos(q3).*cos( ...
  q4).*sin(q2)+cos(q2).*sin(q4))+sin(q2).*sin(q3).*sin(q5)).*sin(q6))+2.*( ...
  cos(q7).*((-1).*cos(q5).*((-1).*cos(q3).*cos(q4).*sin(q2)+cos(q2).*sin( ...
  q4))+(-1).*sin(q2).*sin(q3).*sin(q5))+(-1).*cos(q6).*(cos(q5).*sin(q2).* ...
  sin(q3)+(-1).*((-1).*cos(q3).*cos(q4).*sin(q2)+cos(q2).*sin(q4)).*sin( ...
  q5)).*sin(q7)).^2+2.*(cos(q7).*((-1).*cos(q5).*sin(q2).*sin(q3)+((-1).* ...
  cos(q3).*cos(q4).*sin(q2)+cos(q2).*sin(q4)).*sin(q5))+(-1).*cos(q6).*(( ...
  -1).*cos(q5).*((-1).*cos(q3).*cos(q4).*sin(q2)+cos(q2).*sin(q4))+(-1).* ...
  sin(q2).*sin(q3).*sin(q5)).*sin(q7)).*(cos(q7).*(cos(q5).*sin(q2).*sin( ...
  q3)+(-1).*((-1).*cos(q3).*cos(q4).*sin(q2)+cos(q2).*sin(q4)).*sin(q5))+( ...
  -1).*(cos(q6).*(cos(q5).*((-1).*cos(q3).*cos(q4).*sin(q2)+cos(q2).*sin( ...
  q4))+sin(q2).*sin(q3).*sin(q5))+((-1).*cos(q2).*cos(q4)+(-1).*cos(q3).* ...
  sin(q2).*sin(q4)).*sin(q6)).*sin(q7))).*(((-1).*cos(q6).*((-1).*cos(q2) ...
  .*cos(q4)+(-1).*cos(q3).*sin(q2).*sin(q4))+(cos(q5).*((-1).*cos(q3).* ...
  cos(q4).*sin(q2)+cos(q2).*sin(q4))+sin(q2).*sin(q3).*sin(q5)).*sin(q6)) ...
  .^2+(cos(q7).*(cos(q5).*sin(q2).*sin(q3)+(-1).*((-1).*cos(q3).*cos(q4).* ...
  sin(q2)+cos(q2).*sin(q4)).*sin(q5))+(-1).*(cos(q6).*(cos(q5).*((-1).* ...
  cos(q3).*cos(q4).*sin(q2)+cos(q2).*sin(q4))+sin(q2).*sin(q3).*sin(q5))+( ...
  (-1).*cos(q2).*cos(q4)+(-1).*cos(q3).*sin(q2).*sin(q4)).*sin(q6)).*sin( ...
  q7)).^2).^(-3/2)+(-1).*(cos(q6).*cos(q7).*(cos(q5).*sin(q2).*sin(q3)+( ...
  -1).*((-1).*cos(q3).*cos(q4).*sin(q2)+cos(q2).*sin(q4)).*sin(q5))+((-1) ...
  .*cos(q5).*((-1).*cos(q3).*cos(q4).*sin(q2)+cos(q2).*sin(q4))+(-1).*sin( ...
  q2).*sin(q3).*sin(q5)).*sin(q7)).*(2.*(cos(q5).*sin(q2).*sin(q3)+(-1).*( ...
  (-1).*cos(q3).*cos(q4).*sin(q2)+cos(q2).*sin(q4)).*sin(q5)).*sin(q6).*(( ...
  -1).*cos(q6).*((-1).*cos(q2).*cos(q4)+(-1).*cos(q3).*sin(q2).*sin(q4))+( ...
  cos(q5).*((-1).*cos(q3).*cos(q4).*sin(q2)+cos(q2).*sin(q4))+sin(q2).* ...
  sin(q3).*sin(q5)).*sin(q6))+2.*(cos(q7).*((-1).*cos(q5).*((-1).*cos(q3) ...
  .*cos(q4).*sin(q2)+cos(q2).*sin(q4))+(-1).*sin(q2).*sin(q3).*sin(q5))+( ...
  -1).*cos(q6).*(cos(q5).*sin(q2).*sin(q3)+(-1).*((-1).*cos(q3).*cos(q4).* ...
  sin(q2)+cos(q2).*sin(q4)).*sin(q5)).*sin(q7)).*(cos(q7).*(cos(q5).*sin( ...
  q2).*sin(q3)+(-1).*((-1).*cos(q3).*cos(q4).*sin(q2)+cos(q2).*sin(q4)).* ...
  sin(q5))+(-1).*(cos(q6).*(cos(q5).*((-1).*cos(q3).*cos(q4).*sin(q2)+cos( ...
  q2).*sin(q4))+sin(q2).*sin(q3).*sin(q5))+((-1).*cos(q2).*cos(q4)+(-1).* ...
  cos(q3).*sin(q2).*sin(q4)).*sin(q6)).*sin(q7))).*(((-1).*cos(q6).*((-1) ...
  .*cos(q2).*cos(q4)+(-1).*cos(q3).*sin(q2).*sin(q4))+(cos(q5).*((-1).* ...
  cos(q3).*cos(q4).*sin(q2)+cos(q2).*sin(q4))+sin(q2).*sin(q3).*sin(q5)).* ...
  sin(q6)).^2+(cos(q7).*(cos(q5).*sin(q2).*sin(q3)+(-1).*((-1).*cos(q3).* ...
  cos(q4).*sin(q2)+cos(q2).*sin(q4)).*sin(q5))+(-1).*(cos(q6).*(cos(q5).*( ...
  (-1).*cos(q3).*cos(q4).*sin(q2)+cos(q2).*sin(q4))+sin(q2).*sin(q3).*sin( ...
  q5))+((-1).*cos(q2).*cos(q4)+(-1).*cos(q3).*sin(q2).*sin(q4)).*sin(q6)) ...
  .*sin(q7)).^2).^(-3/2)+(cos(q6).*cos(q7).*((-1).*cos(q5).*((-1).*cos(q3) ...
  .*cos(q4).*sin(q2)+cos(q2).*sin(q4))+(-1).*sin(q2).*sin(q3).*sin(q5))+(( ...
  -1).*cos(q5).*sin(q2).*sin(q3)+((-1).*cos(q3).*cos(q4).*sin(q2)+cos(q2) ...
  .*sin(q4)).*sin(q5)).*sin(q7)).*(((-1).*cos(q6).*((-1).*cos(q2).*cos(q4) ...
  +(-1).*cos(q3).*sin(q2).*sin(q4))+(cos(q5).*((-1).*cos(q3).*cos(q4).* ...
  sin(q2)+cos(q2).*sin(q4))+sin(q2).*sin(q3).*sin(q5)).*sin(q6)).^2+(cos( ...
  q7).*(cos(q5).*sin(q2).*sin(q3)+(-1).*((-1).*cos(q3).*cos(q4).*sin(q2)+ ...
  cos(q2).*sin(q4)).*sin(q5))+(-1).*(cos(q6).*(cos(q5).*((-1).*cos(q3).* ...
  cos(q4).*sin(q2)+cos(q2).*sin(q4))+sin(q2).*sin(q3).*sin(q5))+((-1).* ...
  cos(q2).*cos(q4)+(-1).*cos(q3).*sin(q2).*sin(q4)).*sin(q6)).*sin(q7)) ...
  .^2).^(-1/2));

Jxe256 = (1+(cos(q7).*(cos(q6).*(cos(q5).*((-1).*cos(q3).*cos(q4).* ...
  sin(q2)+cos(q2).*sin(q4))+sin(q2).*sin(q3).*sin(q5))+((-1).*cos(q2).* ...
  cos(q4)+(-1).*cos(q3).*sin(q2).*sin(q4)).*sin(q6))+(cos(q5).*sin(q2).* ...
  sin(q3)+(-1).*((-1).*cos(q3).*cos(q4).*sin(q2)+cos(q2).*sin(q4)).*sin( ...
  q5)).*sin(q7)).^2.*(((-1).*cos(q6).*((-1).*cos(q2).*cos(q4)+(-1).*cos( ...
  q3).*sin(q2).*sin(q4))+(cos(q5).*((-1).*cos(q3).*cos(q4).*sin(q2)+cos( ...
  q2).*sin(q4))+sin(q2).*sin(q3).*sin(q5)).*sin(q6)).^2+(cos(q7).*(cos(q5) ...
  .*sin(q2).*sin(q3)+(-1).*((-1).*cos(q3).*cos(q4).*sin(q2)+cos(q2).*sin( ...
  q4)).*sin(q5))+(-1).*(cos(q6).*(cos(q5).*((-1).*cos(q3).*cos(q4).*sin( ...
  q2)+cos(q2).*sin(q4))+sin(q2).*sin(q3).*sin(q5))+((-1).*cos(q2).*cos(q4) ...
  +(-1).*cos(q3).*sin(q2).*sin(q4)).*sin(q6)).*sin(q7)).^2).^(-1)).^(-1).* ...
  ((3/4).*(cos(q7).*(cos(q6).*(cos(q5).*((-1).*cos(q3).*cos(q4).*sin(q2)+ ...
  cos(q2).*sin(q4))+sin(q2).*sin(q3).*sin(q5))+((-1).*cos(q2).*cos(q4)+( ...
  -1).*cos(q3).*sin(q2).*sin(q4)).*sin(q6))+(cos(q5).*sin(q2).*sin(q3)+( ...
  -1).*((-1).*cos(q3).*cos(q4).*sin(q2)+cos(q2).*sin(q4)).*sin(q5)).*sin( ...
  q7)).*(2.*(cos(q6).*(cos(q5).*((-1).*cos(q3).*cos(q4).*sin(q2)+cos(q2).* ...
  sin(q4))+sin(q2).*sin(q3).*sin(q5))+((-1).*cos(q2).*cos(q4)+(-1).*cos( ...
  q3).*sin(q2).*sin(q4)).*sin(q6)).*((-1).*cos(q6).*((-1).*cos(q2).*cos( ...
  q4)+(-1).*cos(q3).*sin(q2).*sin(q4))+(cos(q5).*((-1).*cos(q3).*cos(q4).* ...
  sin(q2)+cos(q2).*sin(q4))+sin(q2).*sin(q3).*sin(q5)).*sin(q6))+(-2).*( ...
  cos(q6).*((-1).*cos(q2).*cos(q4)+(-1).*cos(q3).*sin(q2).*sin(q4))+(-1).* ...
  (cos(q5).*((-1).*cos(q3).*cos(q4).*sin(q2)+cos(q2).*sin(q4))+sin(q2).* ...
  sin(q3).*sin(q5)).*sin(q6)).*sin(q7).*(cos(q7).*(cos(q5).*sin(q2).*sin( ...
  q3)+(-1).*((-1).*cos(q3).*cos(q4).*sin(q2)+cos(q2).*sin(q4)).*sin(q5))+( ...
  -1).*(cos(q6).*(cos(q5).*((-1).*cos(q3).*cos(q4).*sin(q2)+cos(q2).*sin( ...
  q4))+sin(q2).*sin(q3).*sin(q5))+((-1).*cos(q2).*cos(q4)+(-1).*cos(q3).* ...
  sin(q2).*sin(q4)).*sin(q6)).*sin(q7))).^2.*(((-1).*cos(q6).*((-1).*cos( ...
  q2).*cos(q4)+(-1).*cos(q3).*sin(q2).*sin(q4))+(cos(q5).*((-1).*cos(q3).* ...
  cos(q4).*sin(q2)+cos(q2).*sin(q4))+sin(q2).*sin(q3).*sin(q5)).*sin(q6)) ...
  .^2+(cos(q7).*(cos(q5).*sin(q2).*sin(q3)+(-1).*((-1).*cos(q3).*cos(q4).* ...
  sin(q2)+cos(q2).*sin(q4)).*sin(q5))+(-1).*(cos(q6).*(cos(q5).*((-1).* ...
  cos(q3).*cos(q4).*sin(q2)+cos(q2).*sin(q4))+sin(q2).*sin(q3).*sin(q5))+( ...
  (-1).*cos(q2).*cos(q4)+(-1).*cos(q3).*sin(q2).*sin(q4)).*sin(q6)).*sin( ...
  q7)).^2).^(-5/2)+(-1/2).*(cos(q7).*(cos(q6).*(cos(q5).*((-1).*cos(q3).* ...
  cos(q4).*sin(q2)+cos(q2).*sin(q4))+sin(q2).*sin(q3).*sin(q5))+((-1).* ...
  cos(q2).*cos(q4)+(-1).*cos(q3).*sin(q2).*sin(q4)).*sin(q6))+(cos(q5).* ...
  sin(q2).*sin(q3)+(-1).*((-1).*cos(q3).*cos(q4).*sin(q2)+cos(q2).*sin(q4) ...
  ).*sin(q5)).*sin(q7)).*(2.*(cos(q6).*(cos(q5).*((-1).*cos(q3).*cos(q4).* ...
  sin(q2)+cos(q2).*sin(q4))+sin(q2).*sin(q3).*sin(q5))+((-1).*cos(q2).* ...
  cos(q4)+(-1).*cos(q3).*sin(q2).*sin(q4)).*sin(q6)).^2+2.*(cos(q6).*((-1) ...
  .*cos(q2).*cos(q4)+(-1).*cos(q3).*sin(q2).*sin(q4))+(-1).*(cos(q5).*(( ...
  -1).*cos(q3).*cos(q4).*sin(q2)+cos(q2).*sin(q4))+sin(q2).*sin(q3).*sin( ...
  q5)).*sin(q6)).*((-1).*cos(q6).*((-1).*cos(q2).*cos(q4)+(-1).*cos(q3).* ...
  sin(q2).*sin(q4))+(cos(q5).*((-1).*cos(q3).*cos(q4).*sin(q2)+cos(q2).* ...
  sin(q4))+sin(q2).*sin(q3).*sin(q5)).*sin(q6))+2.*(cos(q6).*((-1).*cos( ...
  q2).*cos(q4)+(-1).*cos(q3).*sin(q2).*sin(q4))+(-1).*(cos(q5).*((-1).* ...
  cos(q3).*cos(q4).*sin(q2)+cos(q2).*sin(q4))+sin(q2).*sin(q3).*sin(q5)).* ...
  sin(q6)).^2.*sin(q7).^2+(-2).*((-1).*cos(q6).*(cos(q5).*((-1).*cos(q3).* ...
  cos(q4).*sin(q2)+cos(q2).*sin(q4))+sin(q2).*sin(q3).*sin(q5))+(-1).*(( ...
  -1).*cos(q2).*cos(q4)+(-1).*cos(q3).*sin(q2).*sin(q4)).*sin(q6)).*sin( ...
  q7).*(cos(q7).*(cos(q5).*sin(q2).*sin(q3)+(-1).*((-1).*cos(q3).*cos(q4) ...
  .*sin(q2)+cos(q2).*sin(q4)).*sin(q5))+(-1).*(cos(q6).*(cos(q5).*((-1).* ...
  cos(q3).*cos(q4).*sin(q2)+cos(q2).*sin(q4))+sin(q2).*sin(q3).*sin(q5))+( ...
  (-1).*cos(q2).*cos(q4)+(-1).*cos(q3).*sin(q2).*sin(q4)).*sin(q6)).*sin( ...
  q7))).*(((-1).*cos(q6).*((-1).*cos(q2).*cos(q4)+(-1).*cos(q3).*sin(q2).* ...
  sin(q4))+(cos(q5).*((-1).*cos(q3).*cos(q4).*sin(q2)+cos(q2).*sin(q4))+ ...
  sin(q2).*sin(q3).*sin(q5)).*sin(q6)).^2+(cos(q7).*(cos(q5).*sin(q2).* ...
  sin(q3)+(-1).*((-1).*cos(q3).*cos(q4).*sin(q2)+cos(q2).*sin(q4)).*sin( ...
  q5))+(-1).*(cos(q6).*(cos(q5).*((-1).*cos(q3).*cos(q4).*sin(q2)+cos(q2) ...
  .*sin(q4))+sin(q2).*sin(q3).*sin(q5))+((-1).*cos(q2).*cos(q4)+(-1).*cos( ...
  q3).*sin(q2).*sin(q4)).*sin(q6)).*sin(q7)).^2).^(-3/2)+(-1).*cos(q7).*( ...
  cos(q6).*((-1).*cos(q2).*cos(q4)+(-1).*cos(q3).*sin(q2).*sin(q4))+(-1).* ...
  (cos(q5).*((-1).*cos(q3).*cos(q4).*sin(q2)+cos(q2).*sin(q4))+sin(q2).* ...
  sin(q3).*sin(q5)).*sin(q6)).*(2.*(cos(q6).*(cos(q5).*((-1).*cos(q3).* ...
  cos(q4).*sin(q2)+cos(q2).*sin(q4))+sin(q2).*sin(q3).*sin(q5))+((-1).* ...
  cos(q2).*cos(q4)+(-1).*cos(q3).*sin(q2).*sin(q4)).*sin(q6)).*((-1).*cos( ...
  q6).*((-1).*cos(q2).*cos(q4)+(-1).*cos(q3).*sin(q2).*sin(q4))+(cos(q5).* ...
  ((-1).*cos(q3).*cos(q4).*sin(q2)+cos(q2).*sin(q4))+sin(q2).*sin(q3).* ...
  sin(q5)).*sin(q6))+(-2).*(cos(q6).*((-1).*cos(q2).*cos(q4)+(-1).*cos(q3) ...
  .*sin(q2).*sin(q4))+(-1).*(cos(q5).*((-1).*cos(q3).*cos(q4).*sin(q2)+ ...
  cos(q2).*sin(q4))+sin(q2).*sin(q3).*sin(q5)).*sin(q6)).*sin(q7).*(cos( ...
  q7).*(cos(q5).*sin(q2).*sin(q3)+(-1).*((-1).*cos(q3).*cos(q4).*sin(q2)+ ...
  cos(q2).*sin(q4)).*sin(q5))+(-1).*(cos(q6).*(cos(q5).*((-1).*cos(q3).* ...
  cos(q4).*sin(q2)+cos(q2).*sin(q4))+sin(q2).*sin(q3).*sin(q5))+((-1).* ...
  cos(q2).*cos(q4)+(-1).*cos(q3).*sin(q2).*sin(q4)).*sin(q6)).*sin(q7))).* ...
  (((-1).*cos(q6).*((-1).*cos(q2).*cos(q4)+(-1).*cos(q3).*sin(q2).*sin(q4) ...
  )+(cos(q5).*((-1).*cos(q3).*cos(q4).*sin(q2)+cos(q2).*sin(q4))+sin(q2).* ...
  sin(q3).*sin(q5)).*sin(q6)).^2+(cos(q7).*(cos(q5).*sin(q2).*sin(q3)+(-1) ...
  .*((-1).*cos(q3).*cos(q4).*sin(q2)+cos(q2).*sin(q4)).*sin(q5))+(-1).*( ...
  cos(q6).*(cos(q5).*((-1).*cos(q3).*cos(q4).*sin(q2)+cos(q2).*sin(q4))+ ...
  sin(q2).*sin(q3).*sin(q5))+((-1).*cos(q2).*cos(q4)+(-1).*cos(q3).*sin( ...
  q2).*sin(q4)).*sin(q6)).*sin(q7)).^2).^(-3/2)+cos(q7).*((-1).*cos(q6).*( ...
  cos(q5).*((-1).*cos(q3).*cos(q4).*sin(q2)+cos(q2).*sin(q4))+sin(q2).* ...
  sin(q3).*sin(q5))+(-1).*((-1).*cos(q2).*cos(q4)+(-1).*cos(q3).*sin(q2).* ...
  sin(q4)).*sin(q6)).*(((-1).*cos(q6).*((-1).*cos(q2).*cos(q4)+(-1).*cos( ...
  q3).*sin(q2).*sin(q4))+(cos(q5).*((-1).*cos(q3).*cos(q4).*sin(q2)+cos( ...
  q2).*sin(q4))+sin(q2).*sin(q3).*sin(q5)).*sin(q6)).^2+(cos(q7).*(cos(q5) ...
  .*sin(q2).*sin(q3)+(-1).*((-1).*cos(q3).*cos(q4).*sin(q2)+cos(q2).*sin( ...
  q4)).*sin(q5))+(-1).*(cos(q6).*(cos(q5).*((-1).*cos(q3).*cos(q4).*sin( ...
  q2)+cos(q2).*sin(q4))+sin(q2).*sin(q3).*sin(q5))+((-1).*cos(q2).*cos(q4) ...
  +(-1).*cos(q3).*sin(q2).*sin(q4)).*sin(q6)).*sin(q7)).^2).^(-1/2))+(-1) ...
  .*((-1).*(cos(q7).*(cos(q6).*(cos(q5).*((-1).*cos(q3).*cos(q4).*sin(q2)+ ...
  cos(q2).*sin(q4))+sin(q2).*sin(q3).*sin(q5))+((-1).*cos(q2).*cos(q4)+( ...
  -1).*cos(q3).*sin(q2).*sin(q4)).*sin(q6))+(cos(q5).*sin(q2).*sin(q3)+( ...
  -1).*((-1).*cos(q3).*cos(q4).*sin(q2)+cos(q2).*sin(q4)).*sin(q5)).*sin( ...
  q7)).^2.*(2.*(cos(q6).*(cos(q5).*((-1).*cos(q3).*cos(q4).*sin(q2)+cos( ...
  q2).*sin(q4))+sin(q2).*sin(q3).*sin(q5))+((-1).*cos(q2).*cos(q4)+(-1).* ...
  cos(q3).*sin(q2).*sin(q4)).*sin(q6)).*((-1).*cos(q6).*((-1).*cos(q2).* ...
  cos(q4)+(-1).*cos(q3).*sin(q2).*sin(q4))+(cos(q5).*((-1).*cos(q3).*cos( ...
  q4).*sin(q2)+cos(q2).*sin(q4))+sin(q2).*sin(q3).*sin(q5)).*sin(q6))+(-2) ...
  .*(cos(q6).*((-1).*cos(q2).*cos(q4)+(-1).*cos(q3).*sin(q2).*sin(q4))+( ...
  -1).*(cos(q5).*((-1).*cos(q3).*cos(q4).*sin(q2)+cos(q2).*sin(q4))+sin( ...
  q2).*sin(q3).*sin(q5)).*sin(q6)).*sin(q7).*(cos(q7).*(cos(q5).*sin(q2).* ...
  sin(q3)+(-1).*((-1).*cos(q3).*cos(q4).*sin(q2)+cos(q2).*sin(q4)).*sin( ...
  q5))+(-1).*(cos(q6).*(cos(q5).*((-1).*cos(q3).*cos(q4).*sin(q2)+cos(q2) ...
  .*sin(q4))+sin(q2).*sin(q3).*sin(q5))+((-1).*cos(q2).*cos(q4)+(-1).*cos( ...
  q3).*sin(q2).*sin(q4)).*sin(q6)).*sin(q7))).*(((-1).*cos(q6).*((-1).* ...
  cos(q2).*cos(q4)+(-1).*cos(q3).*sin(q2).*sin(q4))+(cos(q5).*((-1).*cos( ...
  q3).*cos(q4).*sin(q2)+cos(q2).*sin(q4))+sin(q2).*sin(q3).*sin(q5)).*sin( ...
  q6)).^2+(cos(q7).*(cos(q5).*sin(q2).*sin(q3)+(-1).*((-1).*cos(q3).*cos( ...
  q4).*sin(q2)+cos(q2).*sin(q4)).*sin(q5))+(-1).*(cos(q6).*(cos(q5).*((-1) ...
  .*cos(q3).*cos(q4).*sin(q2)+cos(q2).*sin(q4))+sin(q2).*sin(q3).*sin(q5)) ...
  +((-1).*cos(q2).*cos(q4)+(-1).*cos(q3).*sin(q2).*sin(q4)).*sin(q6)).* ...
  sin(q7)).^2).^(-2)+2.*cos(q7).*(cos(q6).*((-1).*cos(q2).*cos(q4)+(-1).* ...
  cos(q3).*sin(q2).*sin(q4))+(-1).*(cos(q5).*((-1).*cos(q3).*cos(q4).*sin( ...
  q2)+cos(q2).*sin(q4))+sin(q2).*sin(q3).*sin(q5)).*sin(q6)).*(cos(q7).*( ...
  cos(q6).*(cos(q5).*((-1).*cos(q3).*cos(q4).*sin(q2)+cos(q2).*sin(q4))+ ...
  sin(q2).*sin(q3).*sin(q5))+((-1).*cos(q2).*cos(q4)+(-1).*cos(q3).*sin( ...
  q2).*sin(q4)).*sin(q6))+(cos(q5).*sin(q2).*sin(q3)+(-1).*((-1).*cos(q3) ...
  .*cos(q4).*sin(q2)+cos(q2).*sin(q4)).*sin(q5)).*sin(q7)).*(((-1).*cos( ...
  q6).*((-1).*cos(q2).*cos(q4)+(-1).*cos(q3).*sin(q2).*sin(q4))+(cos(q5).* ...
  ((-1).*cos(q3).*cos(q4).*sin(q2)+cos(q2).*sin(q4))+sin(q2).*sin(q3).* ...
  sin(q5)).*sin(q6)).^2+(cos(q7).*(cos(q5).*sin(q2).*sin(q3)+(-1).*((-1).* ...
  cos(q3).*cos(q4).*sin(q2)+cos(q2).*sin(q4)).*sin(q5))+(-1).*(cos(q6).*( ...
  cos(q5).*((-1).*cos(q3).*cos(q4).*sin(q2)+cos(q2).*sin(q4))+sin(q2).* ...
  sin(q3).*sin(q5))+((-1).*cos(q2).*cos(q4)+(-1).*cos(q3).*sin(q2).*sin( ...
  q4)).*sin(q6)).*sin(q7)).^2).^(-1)).*(1+(cos(q7).*(cos(q6).*(cos(q5).*(( ...
  -1).*cos(q3).*cos(q4).*sin(q2)+cos(q2).*sin(q4))+sin(q2).*sin(q3).*sin( ...
  q5))+((-1).*cos(q2).*cos(q4)+(-1).*cos(q3).*sin(q2).*sin(q4)).*sin(q6))+ ...
  (cos(q5).*sin(q2).*sin(q3)+(-1).*((-1).*cos(q3).*cos(q4).*sin(q2)+cos( ...
  q2).*sin(q4)).*sin(q5)).*sin(q7)).^2.*(((-1).*cos(q6).*((-1).*cos(q2).* ...
  cos(q4)+(-1).*cos(q3).*sin(q2).*sin(q4))+(cos(q5).*((-1).*cos(q3).*cos( ...
  q4).*sin(q2)+cos(q2).*sin(q4))+sin(q2).*sin(q3).*sin(q5)).*sin(q6)).^2+( ...
  cos(q7).*(cos(q5).*sin(q2).*sin(q3)+(-1).*((-1).*cos(q3).*cos(q4).*sin( ...
  q2)+cos(q2).*sin(q4)).*sin(q5))+(-1).*(cos(q6).*(cos(q5).*((-1).*cos(q3) ...
  .*cos(q4).*sin(q2)+cos(q2).*sin(q4))+sin(q2).*sin(q3).*sin(q5))+((-1).* ...
  cos(q2).*cos(q4)+(-1).*cos(q3).*sin(q2).*sin(q4)).*sin(q6)).*sin(q7)) ...
  .^2).^(-1)).^(-2).*((-1/2).*(cos(q7).*(cos(q6).*(cos(q5).*((-1).*cos(q3) ...
  .*cos(q4).*sin(q2)+cos(q2).*sin(q4))+sin(q2).*sin(q3).*sin(q5))+((-1).* ...
  cos(q2).*cos(q4)+(-1).*cos(q3).*sin(q2).*sin(q4)).*sin(q6))+(cos(q5).* ...
  sin(q2).*sin(q3)+(-1).*((-1).*cos(q3).*cos(q4).*sin(q2)+cos(q2).*sin(q4) ...
  ).*sin(q5)).*sin(q7)).*(2.*(cos(q6).*(cos(q5).*((-1).*cos(q3).*cos(q4).* ...
  sin(q2)+cos(q2).*sin(q4))+sin(q2).*sin(q3).*sin(q5))+((-1).*cos(q2).* ...
  cos(q4)+(-1).*cos(q3).*sin(q2).*sin(q4)).*sin(q6)).*((-1).*cos(q6).*(( ...
  -1).*cos(q2).*cos(q4)+(-1).*cos(q3).*sin(q2).*sin(q4))+(cos(q5).*((-1).* ...
  cos(q3).*cos(q4).*sin(q2)+cos(q2).*sin(q4))+sin(q2).*sin(q3).*sin(q5)).* ...
  sin(q6))+(-2).*(cos(q6).*((-1).*cos(q2).*cos(q4)+(-1).*cos(q3).*sin(q2) ...
  .*sin(q4))+(-1).*(cos(q5).*((-1).*cos(q3).*cos(q4).*sin(q2)+cos(q2).* ...
  sin(q4))+sin(q2).*sin(q3).*sin(q5)).*sin(q6)).*sin(q7).*(cos(q7).*(cos( ...
  q5).*sin(q2).*sin(q3)+(-1).*((-1).*cos(q3).*cos(q4).*sin(q2)+cos(q2).* ...
  sin(q4)).*sin(q5))+(-1).*(cos(q6).*(cos(q5).*((-1).*cos(q3).*cos(q4).* ...
  sin(q2)+cos(q2).*sin(q4))+sin(q2).*sin(q3).*sin(q5))+((-1).*cos(q2).* ...
  cos(q4)+(-1).*cos(q3).*sin(q2).*sin(q4)).*sin(q6)).*sin(q7))).*(((-1).* ...
  cos(q6).*((-1).*cos(q2).*cos(q4)+(-1).*cos(q3).*sin(q2).*sin(q4))+(cos( ...
  q5).*((-1).*cos(q3).*cos(q4).*sin(q2)+cos(q2).*sin(q4))+sin(q2).*sin(q3) ...
  .*sin(q5)).*sin(q6)).^2+(cos(q7).*(cos(q5).*sin(q2).*sin(q3)+(-1).*((-1) ...
  .*cos(q3).*cos(q4).*sin(q2)+cos(q2).*sin(q4)).*sin(q5))+(-1).*(cos(q6).* ...
  (cos(q5).*((-1).*cos(q3).*cos(q4).*sin(q2)+cos(q2).*sin(q4))+sin(q2).* ...
  sin(q3).*sin(q5))+((-1).*cos(q2).*cos(q4)+(-1).*cos(q3).*sin(q2).*sin( ...
  q4)).*sin(q6)).*sin(q7)).^2).^(-3/2)+cos(q7).*(cos(q6).*((-1).*cos(q2).* ...
  cos(q4)+(-1).*cos(q3).*sin(q2).*sin(q4))+(-1).*(cos(q5).*((-1).*cos(q3) ...
  .*cos(q4).*sin(q2)+cos(q2).*sin(q4))+sin(q2).*sin(q3).*sin(q5)).*sin(q6) ...
  ).*(((-1).*cos(q6).*((-1).*cos(q2).*cos(q4)+(-1).*cos(q3).*sin(q2).*sin( ...
  q4))+(cos(q5).*((-1).*cos(q3).*cos(q4).*sin(q2)+cos(q2).*sin(q4))+sin( ...
  q2).*sin(q3).*sin(q5)).*sin(q6)).^2+(cos(q7).*(cos(q5).*sin(q2).*sin(q3) ...
  +(-1).*((-1).*cos(q3).*cos(q4).*sin(q2)+cos(q2).*sin(q4)).*sin(q5))+(-1) ...
  .*(cos(q6).*(cos(q5).*((-1).*cos(q3).*cos(q4).*sin(q2)+cos(q2).*sin(q4)) ...
  +sin(q2).*sin(q3).*sin(q5))+((-1).*cos(q2).*cos(q4)+(-1).*cos(q3).*sin( ...
  q2).*sin(q4)).*sin(q6)).*sin(q7)).^2).^(-1/2));

Jxe257 = (1+(cos(q7).*(cos(q6).*( ...
  cos(q5).*((-1).*cos(q3).*cos(q4).*sin(q2)+cos(q2).*sin(q4))+sin(q2).* ...
  sin(q3).*sin(q5))+((-1).*cos(q2).*cos(q4)+(-1).*cos(q3).*sin(q2).*sin( ...
  q4)).*sin(q6))+(cos(q5).*sin(q2).*sin(q3)+(-1).*((-1).*cos(q3).*cos(q4) ...
  .*sin(q2)+cos(q2).*sin(q4)).*sin(q5)).*sin(q7)).^2.*(((-1).*cos(q6).*(( ...
  -1).*cos(q2).*cos(q4)+(-1).*cos(q3).*sin(q2).*sin(q4))+(cos(q5).*((-1).* ...
  cos(q3).*cos(q4).*sin(q2)+cos(q2).*sin(q4))+sin(q2).*sin(q3).*sin(q5)).* ...
  sin(q6)).^2+(cos(q7).*(cos(q5).*sin(q2).*sin(q3)+(-1).*((-1).*cos(q3).* ...
  cos(q4).*sin(q2)+cos(q2).*sin(q4)).*sin(q5))+(-1).*(cos(q6).*(cos(q5).*( ...
  (-1).*cos(q3).*cos(q4).*sin(q2)+cos(q2).*sin(q4))+sin(q2).*sin(q3).*sin( ...
  q5))+((-1).*cos(q2).*cos(q4)+(-1).*cos(q3).*sin(q2).*sin(q4)).*sin(q6)) ...
  .*sin(q7)).^2).^(-1)).^(-1).*(3.*((-1).*cos(q7).*(cos(q6).*(cos(q5).*(( ...
  -1).*cos(q3).*cos(q4).*sin(q2)+cos(q2).*sin(q4))+sin(q2).*sin(q3).*sin( ...
  q5))+((-1).*cos(q2).*cos(q4)+(-1).*cos(q3).*sin(q2).*sin(q4)).*sin(q6))+ ...
  (-1).*(cos(q5).*sin(q2).*sin(q3)+(-1).*((-1).*cos(q3).*cos(q4).*sin(q2)+ ...
  cos(q2).*sin(q4)).*sin(q5)).*sin(q7)).^2.*(cos(q7).*(cos(q6).*(cos(q5).* ...
  ((-1).*cos(q3).*cos(q4).*sin(q2)+cos(q2).*sin(q4))+sin(q2).*sin(q3).* ...
  sin(q5))+((-1).*cos(q2).*cos(q4)+(-1).*cos(q3).*sin(q2).*sin(q4)).*sin( ...
  q6))+(cos(q5).*sin(q2).*sin(q3)+(-1).*((-1).*cos(q3).*cos(q4).*sin(q2)+ ...
  cos(q2).*sin(q4)).*sin(q5)).*sin(q7)).*(cos(q7).*(cos(q5).*sin(q2).*sin( ...
  q3)+(-1).*((-1).*cos(q3).*cos(q4).*sin(q2)+cos(q2).*sin(q4)).*sin(q5))+( ...
  -1).*(cos(q6).*(cos(q5).*((-1).*cos(q3).*cos(q4).*sin(q2)+cos(q2).*sin( ...
  q4))+sin(q2).*sin(q3).*sin(q5))+((-1).*cos(q2).*cos(q4)+(-1).*cos(q3).* ...
  sin(q2).*sin(q4)).*sin(q6)).*sin(q7)).^2.*(((-1).*cos(q6).*((-1).*cos( ...
  q2).*cos(q4)+(-1).*cos(q3).*sin(q2).*sin(q4))+(cos(q5).*((-1).*cos(q3).* ...
  cos(q4).*sin(q2)+cos(q2).*sin(q4))+sin(q2).*sin(q3).*sin(q5)).*sin(q6)) ...
  .^2+(cos(q7).*(cos(q5).*sin(q2).*sin(q3)+(-1).*((-1).*cos(q3).*cos(q4).* ...
  sin(q2)+cos(q2).*sin(q4)).*sin(q5))+(-1).*(cos(q6).*(cos(q5).*((-1).* ...
  cos(q3).*cos(q4).*sin(q2)+cos(q2).*sin(q4))+sin(q2).*sin(q3).*sin(q5))+( ...
  (-1).*cos(q2).*cos(q4)+(-1).*cos(q3).*sin(q2).*sin(q4)).*sin(q6)).*sin( ...
  q7)).^2).^(-5/2)+(-1).*((-1).*cos(q7).*(cos(q6).*(cos(q5).*((-1).*cos( ...
  q3).*cos(q4).*sin(q2)+cos(q2).*sin(q4))+sin(q2).*sin(q3).*sin(q5))+((-1) ...
  .*cos(q2).*cos(q4)+(-1).*cos(q3).*sin(q2).*sin(q4)).*sin(q6))+(-1).*( ...
  cos(q5).*sin(q2).*sin(q3)+(-1).*((-1).*cos(q3).*cos(q4).*sin(q2)+cos(q2) ...
  .*sin(q4)).*sin(q5)).*sin(q7)).^2.*(cos(q7).*(cos(q6).*(cos(q5).*((-1).* ...
  cos(q3).*cos(q4).*sin(q2)+cos(q2).*sin(q4))+sin(q2).*sin(q3).*sin(q5))+( ...
  (-1).*cos(q2).*cos(q4)+(-1).*cos(q3).*sin(q2).*sin(q4)).*sin(q6))+(cos( ...
  q5).*sin(q2).*sin(q3)+(-1).*((-1).*cos(q3).*cos(q4).*sin(q2)+cos(q2).* ...
  sin(q4)).*sin(q5)).*sin(q7)).*(((-1).*cos(q6).*((-1).*cos(q2).*cos(q4)+( ...
  -1).*cos(q3).*sin(q2).*sin(q4))+(cos(q5).*((-1).*cos(q3).*cos(q4).*sin( ...
  q2)+cos(q2).*sin(q4))+sin(q2).*sin(q3).*sin(q5)).*sin(q6)).^2+(cos(q7).* ...
  (cos(q5).*sin(q2).*sin(q3)+(-1).*((-1).*cos(q3).*cos(q4).*sin(q2)+cos( ...
  q2).*sin(q4)).*sin(q5))+(-1).*(cos(q6).*(cos(q5).*((-1).*cos(q3).*cos( ...
  q4).*sin(q2)+cos(q2).*sin(q4))+sin(q2).*sin(q3).*sin(q5))+((-1).*cos(q2) ...
  .*cos(q4)+(-1).*cos(q3).*sin(q2).*sin(q4)).*sin(q6)).*sin(q7)).^2).^( ...
  -3/2)+(-2).*((-1).*cos(q7).*(cos(q6).*(cos(q5).*((-1).*cos(q3).*cos(q4) ...
  .*sin(q2)+cos(q2).*sin(q4))+sin(q2).*sin(q3).*sin(q5))+((-1).*cos(q2).* ...
  cos(q4)+(-1).*cos(q3).*sin(q2).*sin(q4)).*sin(q6))+(-1).*(cos(q5).*sin( ...
  q2).*sin(q3)+(-1).*((-1).*cos(q3).*cos(q4).*sin(q2)+cos(q2).*sin(q4)).* ...
  sin(q5)).*sin(q7)).*(cos(q7).*(cos(q5).*sin(q2).*sin(q3)+(-1).*((-1).* ...
  cos(q3).*cos(q4).*sin(q2)+cos(q2).*sin(q4)).*sin(q5))+(-1).*(cos(q6).*( ...
  cos(q5).*((-1).*cos(q3).*cos(q4).*sin(q2)+cos(q2).*sin(q4))+sin(q2).* ...
  sin(q3).*sin(q5))+((-1).*cos(q2).*cos(q4)+(-1).*cos(q3).*sin(q2).*sin( ...
  q4)).*sin(q6)).*sin(q7)).^2.*(((-1).*cos(q6).*((-1).*cos(q2).*cos(q4)+( ...
  -1).*cos(q3).*sin(q2).*sin(q4))+(cos(q5).*((-1).*cos(q3).*cos(q4).*sin( ...
  q2)+cos(q2).*sin(q4))+sin(q2).*sin(q3).*sin(q5)).*sin(q6)).^2+(cos(q7).* ...
  (cos(q5).*sin(q2).*sin(q3)+(-1).*((-1).*cos(q3).*cos(q4).*sin(q2)+cos( ...
  q2).*sin(q4)).*sin(q5))+(-1).*(cos(q6).*(cos(q5).*((-1).*cos(q3).*cos( ...
  q4).*sin(q2)+cos(q2).*sin(q4))+sin(q2).*sin(q3).*sin(q5))+((-1).*cos(q2) ...
  .*cos(q4)+(-1).*cos(q3).*sin(q2).*sin(q4)).*sin(q6)).*sin(q7)).^2).^( ...
  -3/2)+(-1).*(cos(q7).*(cos(q6).*(cos(q5).*((-1).*cos(q3).*cos(q4).*sin( ...
  q2)+cos(q2).*sin(q4))+sin(q2).*sin(q3).*sin(q5))+((-1).*cos(q2).*cos(q4) ...
  +(-1).*cos(q3).*sin(q2).*sin(q4)).*sin(q6))+(cos(q5).*sin(q2).*sin(q3)+( ...
  -1).*((-1).*cos(q3).*cos(q4).*sin(q2)+cos(q2).*sin(q4)).*sin(q5)).*sin( ...
  q7)).*(cos(q7).*(cos(q5).*sin(q2).*sin(q3)+(-1).*((-1).*cos(q3).*cos(q4) ...
  .*sin(q2)+cos(q2).*sin(q4)).*sin(q5))+(-1).*(cos(q6).*(cos(q5).*((-1).* ...
  cos(q3).*cos(q4).*sin(q2)+cos(q2).*sin(q4))+sin(q2).*sin(q3).*sin(q5))+( ...
  (-1).*cos(q2).*cos(q4)+(-1).*cos(q3).*sin(q2).*sin(q4)).*sin(q6)).*sin( ...
  q7)).*((-1).*cos(q7).*(cos(q5).*sin(q2).*sin(q3)+(-1).*((-1).*cos(q3).* ...
  cos(q4).*sin(q2)+cos(q2).*sin(q4)).*sin(q5))+(cos(q6).*(cos(q5).*((-1).* ...
  cos(q3).*cos(q4).*sin(q2)+cos(q2).*sin(q4))+sin(q2).*sin(q3).*sin(q5))+( ...
  (-1).*cos(q2).*cos(q4)+(-1).*cos(q3).*sin(q2).*sin(q4)).*sin(q6)).*sin( ...
  q7)).*(((-1).*cos(q6).*((-1).*cos(q2).*cos(q4)+(-1).*cos(q3).*sin(q2).* ...
  sin(q4))+(cos(q5).*((-1).*cos(q3).*cos(q4).*sin(q2)+cos(q2).*sin(q4))+ ...
  sin(q2).*sin(q3).*sin(q5)).*sin(q6)).^2+(cos(q7).*(cos(q5).*sin(q2).* ...
  sin(q3)+(-1).*((-1).*cos(q3).*cos(q4).*sin(q2)+cos(q2).*sin(q4)).*sin( ...
  q5))+(-1).*(cos(q6).*(cos(q5).*((-1).*cos(q3).*cos(q4).*sin(q2)+cos(q2) ...
  .*sin(q4))+sin(q2).*sin(q3).*sin(q5))+((-1).*cos(q2).*cos(q4)+(-1).*cos( ...
  q3).*sin(q2).*sin(q4)).*sin(q6)).*sin(q7)).^2).^(-3/2)+((-1).*cos(q7).*( ...
  cos(q6).*(cos(q5).*((-1).*cos(q3).*cos(q4).*sin(q2)+cos(q2).*sin(q4))+ ...
  sin(q2).*sin(q3).*sin(q5))+((-1).*cos(q2).*cos(q4)+(-1).*cos(q3).*sin( ...
  q2).*sin(q4)).*sin(q6))+(-1).*(cos(q5).*sin(q2).*sin(q3)+(-1).*((-1).* ...
  cos(q3).*cos(q4).*sin(q2)+cos(q2).*sin(q4)).*sin(q5)).*sin(q7)).*(((-1) ...
  .*cos(q6).*((-1).*cos(q2).*cos(q4)+(-1).*cos(q3).*sin(q2).*sin(q4))+( ...
  cos(q5).*((-1).*cos(q3).*cos(q4).*sin(q2)+cos(q2).*sin(q4))+sin(q2).* ...
  sin(q3).*sin(q5)).*sin(q6)).^2+(cos(q7).*(cos(q5).*sin(q2).*sin(q3)+(-1) ...
  .*((-1).*cos(q3).*cos(q4).*sin(q2)+cos(q2).*sin(q4)).*sin(q5))+(-1).*( ...
  cos(q6).*(cos(q5).*((-1).*cos(q3).*cos(q4).*sin(q2)+cos(q2).*sin(q4))+ ...
  sin(q2).*sin(q3).*sin(q5))+((-1).*cos(q2).*cos(q4)+(-1).*cos(q3).*sin( ...
  q2).*sin(q4)).*sin(q6)).*sin(q7)).^2).^(-1/2))+(-1).*(1+(cos(q7).*(cos( ...
  q6).*(cos(q5).*((-1).*cos(q3).*cos(q4).*sin(q2)+cos(q2).*sin(q4))+sin( ...
  q2).*sin(q3).*sin(q5))+((-1).*cos(q2).*cos(q4)+(-1).*cos(q3).*sin(q2).* ...
  sin(q4)).*sin(q6))+(cos(q5).*sin(q2).*sin(q3)+(-1).*((-1).*cos(q3).*cos( ...
  q4).*sin(q2)+cos(q2).*sin(q4)).*sin(q5)).*sin(q7)).^2.*(((-1).*cos(q6).* ...
  ((-1).*cos(q2).*cos(q4)+(-1).*cos(q3).*sin(q2).*sin(q4))+(cos(q5).*((-1) ...
  .*cos(q3).*cos(q4).*sin(q2)+cos(q2).*sin(q4))+sin(q2).*sin(q3).*sin(q5)) ...
  .*sin(q6)).^2+(cos(q7).*(cos(q5).*sin(q2).*sin(q3)+(-1).*((-1).*cos(q3) ...
  .*cos(q4).*sin(q2)+cos(q2).*sin(q4)).*sin(q5))+(-1).*(cos(q6).*(cos(q5) ...
  .*((-1).*cos(q3).*cos(q4).*sin(q2)+cos(q2).*sin(q4))+sin(q2).*sin(q3).* ...
  sin(q5))+((-1).*cos(q2).*cos(q4)+(-1).*cos(q3).*sin(q2).*sin(q4)).*sin( ...
  q6)).*sin(q7)).^2).^(-1)).^(-2).*((-2).*((-1).*cos(q7).*(cos(q6).*(cos( ...
  q5).*((-1).*cos(q3).*cos(q4).*sin(q2)+cos(q2).*sin(q4))+sin(q2).*sin(q3) ...
  .*sin(q5))+((-1).*cos(q2).*cos(q4)+(-1).*cos(q3).*sin(q2).*sin(q4)).* ...
  sin(q6))+(-1).*(cos(q5).*sin(q2).*sin(q3)+(-1).*((-1).*cos(q3).*cos(q4) ...
  .*sin(q2)+cos(q2).*sin(q4)).*sin(q5)).*sin(q7)).*(cos(q7).*(cos(q6).*( ...
  cos(q5).*((-1).*cos(q3).*cos(q4).*sin(q2)+cos(q2).*sin(q4))+sin(q2).* ...
  sin(q3).*sin(q5))+((-1).*cos(q2).*cos(q4)+(-1).*cos(q3).*sin(q2).*sin( ...
  q4)).*sin(q6))+(cos(q5).*sin(q2).*sin(q3)+(-1).*((-1).*cos(q3).*cos(q4) ...
  .*sin(q2)+cos(q2).*sin(q4)).*sin(q5)).*sin(q7)).^2.*(cos(q7).*(cos(q5).* ...
  sin(q2).*sin(q3)+(-1).*((-1).*cos(q3).*cos(q4).*sin(q2)+cos(q2).*sin(q4) ...
  ).*sin(q5))+(-1).*(cos(q6).*(cos(q5).*((-1).*cos(q3).*cos(q4).*sin(q2)+ ...
  cos(q2).*sin(q4))+sin(q2).*sin(q3).*sin(q5))+((-1).*cos(q2).*cos(q4)+( ...
  -1).*cos(q3).*sin(q2).*sin(q4)).*sin(q6)).*sin(q7)).*(((-1).*cos(q6).*(( ...
  -1).*cos(q2).*cos(q4)+(-1).*cos(q3).*sin(q2).*sin(q4))+(cos(q5).*((-1).* ...
  cos(q3).*cos(q4).*sin(q2)+cos(q2).*sin(q4))+sin(q2).*sin(q3).*sin(q5)).* ...
  sin(q6)).^2+(cos(q7).*(cos(q5).*sin(q2).*sin(q3)+(-1).*((-1).*cos(q3).* ...
  cos(q4).*sin(q2)+cos(q2).*sin(q4)).*sin(q5))+(-1).*(cos(q6).*(cos(q5).*( ...
  (-1).*cos(q3).*cos(q4).*sin(q2)+cos(q2).*sin(q4))+sin(q2).*sin(q3).*sin( ...
  q5))+((-1).*cos(q2).*cos(q4)+(-1).*cos(q3).*sin(q2).*sin(q4)).*sin(q6)) ...
  .*sin(q7)).^2).^(-2)+2.*(cos(q7).*(cos(q6).*(cos(q5).*((-1).*cos(q3).* ...
  cos(q4).*sin(q2)+cos(q2).*sin(q4))+sin(q2).*sin(q3).*sin(q5))+((-1).* ...
  cos(q2).*cos(q4)+(-1).*cos(q3).*sin(q2).*sin(q4)).*sin(q6))+(cos(q5).* ...
  sin(q2).*sin(q3)+(-1).*((-1).*cos(q3).*cos(q4).*sin(q2)+cos(q2).*sin(q4) ...
  ).*sin(q5)).*sin(q7)).*(cos(q7).*(cos(q5).*sin(q2).*sin(q3)+(-1).*((-1) ...
  .*cos(q3).*cos(q4).*sin(q2)+cos(q2).*sin(q4)).*sin(q5))+(-1).*(cos(q6).* ...
  (cos(q5).*((-1).*cos(q3).*cos(q4).*sin(q2)+cos(q2).*sin(q4))+sin(q2).* ...
  sin(q3).*sin(q5))+((-1).*cos(q2).*cos(q4)+(-1).*cos(q3).*sin(q2).*sin( ...
  q4)).*sin(q6)).*sin(q7)).*(((-1).*cos(q6).*((-1).*cos(q2).*cos(q4)+(-1) ...
  .*cos(q3).*sin(q2).*sin(q4))+(cos(q5).*((-1).*cos(q3).*cos(q4).*sin(q2)+ ...
  cos(q2).*sin(q4))+sin(q2).*sin(q3).*sin(q5)).*sin(q6)).^2+(cos(q7).*( ...
  cos(q5).*sin(q2).*sin(q3)+(-1).*((-1).*cos(q3).*cos(q4).*sin(q2)+cos(q2) ...
  .*sin(q4)).*sin(q5))+(-1).*(cos(q6).*(cos(q5).*((-1).*cos(q3).*cos(q4).* ...
  sin(q2)+cos(q2).*sin(q4))+sin(q2).*sin(q3).*sin(q5))+((-1).*cos(q2).* ...
  cos(q4)+(-1).*cos(q3).*sin(q2).*sin(q4)).*sin(q6)).*sin(q7)).^2).^(-1)) ...
  .*((-1).*((-1).*cos(q7).*(cos(q6).*(cos(q5).*((-1).*cos(q3).*cos(q4).* ...
  sin(q2)+cos(q2).*sin(q4))+sin(q2).*sin(q3).*sin(q5))+((-1).*cos(q2).* ...
  cos(q4)+(-1).*cos(q3).*sin(q2).*sin(q4)).*sin(q6))+(-1).*(cos(q5).*sin( ...
  q2).*sin(q3)+(-1).*((-1).*cos(q3).*cos(q4).*sin(q2)+cos(q2).*sin(q4)).* ...
  sin(q5)).*sin(q7)).*(cos(q7).*(cos(q6).*(cos(q5).*((-1).*cos(q3).*cos( ...
  q4).*sin(q2)+cos(q2).*sin(q4))+sin(q2).*sin(q3).*sin(q5))+((-1).*cos(q2) ...
  .*cos(q4)+(-1).*cos(q3).*sin(q2).*sin(q4)).*sin(q6))+(cos(q5).*sin(q2).* ...
  sin(q3)+(-1).*((-1).*cos(q3).*cos(q4).*sin(q2)+cos(q2).*sin(q4)).*sin( ...
  q5)).*sin(q7)).*(cos(q7).*(cos(q5).*sin(q2).*sin(q3)+(-1).*((-1).*cos( ...
  q3).*cos(q4).*sin(q2)+cos(q2).*sin(q4)).*sin(q5))+(-1).*(cos(q6).*(cos( ...
  q5).*((-1).*cos(q3).*cos(q4).*sin(q2)+cos(q2).*sin(q4))+sin(q2).*sin(q3) ...
  .*sin(q5))+((-1).*cos(q2).*cos(q4)+(-1).*cos(q3).*sin(q2).*sin(q4)).* ...
  sin(q6)).*sin(q7)).*(((-1).*cos(q6).*((-1).*cos(q2).*cos(q4)+(-1).*cos( ...
  q3).*sin(q2).*sin(q4))+(cos(q5).*((-1).*cos(q3).*cos(q4).*sin(q2)+cos( ...
  q2).*sin(q4))+sin(q2).*sin(q3).*sin(q5)).*sin(q6)).^2+(cos(q7).*(cos(q5) ...
  .*sin(q2).*sin(q3)+(-1).*((-1).*cos(q3).*cos(q4).*sin(q2)+cos(q2).*sin( ...
  q4)).*sin(q5))+(-1).*(cos(q6).*(cos(q5).*((-1).*cos(q3).*cos(q4).*sin( ...
  q2)+cos(q2).*sin(q4))+sin(q2).*sin(q3).*sin(q5))+((-1).*cos(q2).*cos(q4) ...
  +(-1).*cos(q3).*sin(q2).*sin(q4)).*sin(q6)).*sin(q7)).^2).^(-3/2)+(cos( ...
  q7).*(cos(q5).*sin(q2).*sin(q3)+(-1).*((-1).*cos(q3).*cos(q4).*sin(q2)+ ...
  cos(q2).*sin(q4)).*sin(q5))+(-1).*(cos(q6).*(cos(q5).*((-1).*cos(q3).* ...
  cos(q4).*sin(q2)+cos(q2).*sin(q4))+sin(q2).*sin(q3).*sin(q5))+((-1).* ...
  cos(q2).*cos(q4)+(-1).*cos(q3).*sin(q2).*sin(q4)).*sin(q6)).*sin(q7)).*( ...
  ((-1).*cos(q6).*((-1).*cos(q2).*cos(q4)+(-1).*cos(q3).*sin(q2).*sin(q4)) ...
  +(cos(q5).*((-1).*cos(q3).*cos(q4).*sin(q2)+cos(q2).*sin(q4))+sin(q2).* ...
  sin(q3).*sin(q5)).*sin(q6)).^2+(cos(q7).*(cos(q5).*sin(q2).*sin(q3)+(-1) ...
  .*((-1).*cos(q3).*cos(q4).*sin(q2)+cos(q2).*sin(q4)).*sin(q5))+(-1).*( ...
  cos(q6).*(cos(q5).*((-1).*cos(q3).*cos(q4).*sin(q2)+cos(q2).*sin(q4))+ ...
  sin(q2).*sin(q3).*sin(q5))+((-1).*cos(q2).*cos(q4)+(-1).*cos(q3).*sin( ...
  q2).*sin(q4)).*sin(q6)).*sin(q7)).^2).^(-1/2));

Jxe261 = 0;

Jxe262 = (-2).*((-1).*cos(q6).*( ...
  cos(q4).*sin(q2)+(-1).*cos(q2).*cos(q3).*sin(q4))+(cos(q5).*((-1).*cos( ...
  q2).*cos(q3).*cos(q4)+(-1).*sin(q2).*sin(q4))+cos(q2).*sin(q3).*sin(q5)) ...
  .*sin(q6)).*((-1).*cos(q6).*((-1).*cos(q2).*cos(q4)+(-1).*cos(q3).*sin( ...
  q2).*sin(q4))+(cos(q5).*((-1).*cos(q3).*cos(q4).*sin(q2)+cos(q2).*sin( ...
  q4))+sin(q2).*sin(q3).*sin(q5)).*sin(q6)).^(-2).*(cos(q7).*(cos(q2).* ...
  cos(q5).*sin(q3)+(-1).*((-1).*cos(q2).*cos(q3).*cos(q4)+(-1).*sin(q2).* ...
  sin(q4)).*sin(q5))+(-1).*(cos(q6).*(cos(q5).*((-1).*cos(q2).*cos(q3).* ...
  cos(q4)+(-1).*sin(q2).*sin(q4))+cos(q2).*sin(q3).*sin(q5))+(cos(q4).* ...
  sin(q2)+(-1).*cos(q2).*cos(q3).*sin(q4)).*sin(q6)).*sin(q7))+(2.*((-1).* ...
  cos(q6).*(cos(q4).*sin(q2)+(-1).*cos(q2).*cos(q3).*sin(q4))+(cos(q5).*(( ...
  -1).*cos(q2).*cos(q3).*cos(q4)+(-1).*sin(q2).*sin(q4))+cos(q2).*sin(q3) ...
  .*sin(q5)).*sin(q6)).^2.*((-1).*cos(q6).*((-1).*cos(q2).*cos(q4)+(-1).* ...
  cos(q3).*sin(q2).*sin(q4))+(cos(q5).*((-1).*cos(q3).*cos(q4).*sin(q2)+ ...
  cos(q2).*sin(q4))+sin(q2).*sin(q3).*sin(q5)).*sin(q6)).^(-3)+(-1).*((-1) ...
  .*cos(q6).*(cos(q2).*cos(q4)+cos(q3).*sin(q2).*sin(q4))+(cos(q5).*(cos( ...
  q3).*cos(q4).*sin(q2)+(-1).*cos(q2).*sin(q4))+(-1).*sin(q2).*sin(q3).* ...
  sin(q5)).*sin(q6)).*((-1).*cos(q6).*((-1).*cos(q2).*cos(q4)+(-1).*cos( ...
  q3).*sin(q2).*sin(q4))+(cos(q5).*((-1).*cos(q3).*cos(q4).*sin(q2)+cos( ...
  q2).*sin(q4))+sin(q2).*sin(q3).*sin(q5)).*sin(q6)).^(-2)).*(cos(q7).*( ...
  cos(q5).*sin(q2).*sin(q3)+(-1).*((-1).*cos(q3).*cos(q4).*sin(q2)+cos(q2) ...
  .*sin(q4)).*sin(q5))+(-1).*(cos(q6).*(cos(q5).*((-1).*cos(q3).*cos(q4).* ...
  sin(q2)+cos(q2).*sin(q4))+sin(q2).*sin(q3).*sin(q5))+((-1).*cos(q2).* ...
  cos(q4)+(-1).*cos(q3).*sin(q2).*sin(q4)).*sin(q6)).*sin(q7))+((-1).*cos( ...
  q6).*((-1).*cos(q2).*cos(q4)+(-1).*cos(q3).*sin(q2).*sin(q4))+(cos(q5).* ...
  ((-1).*cos(q3).*cos(q4).*sin(q2)+cos(q2).*sin(q4))+sin(q2).*sin(q3).* ...
  sin(q5)).*sin(q6)).^(-1).*(cos(q7).*((-1).*cos(q5).*sin(q2).*sin(q3)+(( ...
  -1).*cos(q3).*cos(q4).*sin(q2)+cos(q2).*sin(q4)).*sin(q5))+((-1).*cos( ...
  q6).*(cos(q5).*(cos(q3).*cos(q4).*sin(q2)+(-1).*cos(q2).*sin(q4))+(-1).* ...
  sin(q2).*sin(q3).*sin(q5))+(-1).*(cos(q2).*cos(q4)+cos(q3).*sin(q2).* ...
  sin(q4)).*sin(q6)).*sin(q7));

Jxe263 = ((-1).*cos(q6).*((-1).*cos(q2).*cos(q4)+( ...
  -1).*cos(q3).*sin(q2).*sin(q4))+(cos(q5).*((-1).*cos(q3).*cos(q4).*sin( ...
  q2)+cos(q2).*sin(q4))+sin(q2).*sin(q3).*sin(q5)).*sin(q6)).^(-1).*(cos( ...
  q7).*((-1).*cos(q5).*sin(q2).*sin(q3)+(-1).*cos(q3).*cos(q4).*sin(q2).* ...
  sin(q5))+((-1).*cos(q6).*(cos(q3).*cos(q4).*cos(q5).*sin(q2)+(-1).*sin( ...
  q2).*sin(q3).*sin(q5))+(-1).*cos(q3).*sin(q2).*sin(q4).*sin(q6)).*sin( ...
  q7))+(-2).*((-1).*cos(q6).*sin(q2).*sin(q3).*sin(q4)+(cos(q4).*cos(q5).* ...
  sin(q2).*sin(q3)+cos(q3).*sin(q2).*sin(q5)).*sin(q6)).*((-1).*cos(q6).*( ...
  (-1).*cos(q2).*cos(q4)+(-1).*cos(q3).*sin(q2).*sin(q4))+(cos(q5).*((-1) ...
  .*cos(q3).*cos(q4).*sin(q2)+cos(q2).*sin(q4))+sin(q2).*sin(q3).*sin(q5)) ...
  .*sin(q6)).^(-2).*(cos(q7).*(cos(q3).*cos(q5).*sin(q2)+(-1).*cos(q4).* ...
  sin(q2).*sin(q3).*sin(q5))+(-1).*(cos(q6).*(cos(q4).*cos(q5).*sin(q2).* ...
  sin(q3)+cos(q3).*sin(q2).*sin(q5))+sin(q2).*sin(q3).*sin(q4).*sin(q6)).* ...
  sin(q7))+(2.*((-1).*cos(q6).*sin(q2).*sin(q3).*sin(q4)+(cos(q4).*cos(q5) ...
  .*sin(q2).*sin(q3)+cos(q3).*sin(q2).*sin(q5)).*sin(q6)).^2.*((-1).*cos( ...
  q6).*((-1).*cos(q2).*cos(q4)+(-1).*cos(q3).*sin(q2).*sin(q4))+(cos(q5).* ...
  ((-1).*cos(q3).*cos(q4).*sin(q2)+cos(q2).*sin(q4))+sin(q2).*sin(q3).* ...
  sin(q5)).*sin(q6)).^(-3)+(-1).*((-1).*cos(q3).*cos(q6).*sin(q2).*sin(q4) ...
  +(cos(q3).*cos(q4).*cos(q5).*sin(q2)+(-1).*sin(q2).*sin(q3).*sin(q5)).* ...
  sin(q6)).*((-1).*cos(q6).*((-1).*cos(q2).*cos(q4)+(-1).*cos(q3).*sin(q2) ...
  .*sin(q4))+(cos(q5).*((-1).*cos(q3).*cos(q4).*sin(q2)+cos(q2).*sin(q4))+ ...
  sin(q2).*sin(q3).*sin(q5)).*sin(q6)).^(-2)).*(cos(q7).*(cos(q5).*sin(q2) ...
  .*sin(q3)+(-1).*((-1).*cos(q3).*cos(q4).*sin(q2)+cos(q2).*sin(q4)).*sin( ...
  q5))+(-1).*(cos(q6).*(cos(q5).*((-1).*cos(q3).*cos(q4).*sin(q2)+cos(q2) ...
  .*sin(q4))+sin(q2).*sin(q3).*sin(q5))+((-1).*cos(q2).*cos(q4)+(-1).*cos( ...
  q3).*sin(q2).*sin(q4)).*sin(q6)).*sin(q7));

Jxe264 = (-2).*((-1).*cos(q6).*((-1).* ...
  cos(q3).*cos(q4).*sin(q2)+cos(q2).*sin(q4))+cos(q5).*(cos(q2).*cos(q4)+ ...
  cos(q3).*sin(q2).*sin(q4)).*sin(q6)).*((-1).*cos(q6).*((-1).*cos(q2).* ...
  cos(q4)+(-1).*cos(q3).*sin(q2).*sin(q4))+(cos(q5).*((-1).*cos(q3).*cos( ...
  q4).*sin(q2)+cos(q2).*sin(q4))+sin(q2).*sin(q3).*sin(q5)).*sin(q6)).^( ...
  -2).*((-1).*cos(q7).*(cos(q2).*cos(q4)+cos(q3).*sin(q2).*sin(q4)).*sin( ...
  q5)+(-1).*(cos(q5).*cos(q6).*(cos(q2).*cos(q4)+cos(q3).*sin(q2).*sin(q4) ...
  )+((-1).*cos(q3).*cos(q4).*sin(q2)+cos(q2).*sin(q4)).*sin(q6)).*sin(q7)) ...
  +(2.*((-1).*cos(q6).*((-1).*cos(q3).*cos(q4).*sin(q2)+cos(q2).*sin(q4))+ ...
  cos(q5).*(cos(q2).*cos(q4)+cos(q3).*sin(q2).*sin(q4)).*sin(q6)).^2.*(( ...
  -1).*cos(q6).*((-1).*cos(q2).*cos(q4)+(-1).*cos(q3).*sin(q2).*sin(q4))+( ...
  cos(q5).*((-1).*cos(q3).*cos(q4).*sin(q2)+cos(q2).*sin(q4))+sin(q2).* ...
  sin(q3).*sin(q5)).*sin(q6)).^(-3)+(-1).*((-1).*cos(q6).*(cos(q2).*cos( ...
  q4)+cos(q3).*sin(q2).*sin(q4))+cos(q5).*(cos(q3).*cos(q4).*sin(q2)+(-1) ...
  .*cos(q2).*sin(q4)).*sin(q6)).*((-1).*cos(q6).*((-1).*cos(q2).*cos(q4)+( ...
  -1).*cos(q3).*sin(q2).*sin(q4))+(cos(q5).*((-1).*cos(q3).*cos(q4).*sin( ...
  q2)+cos(q2).*sin(q4))+sin(q2).*sin(q3).*sin(q5)).*sin(q6)).^(-2)).*(cos( ...
  q7).*(cos(q5).*sin(q2).*sin(q3)+(-1).*((-1).*cos(q3).*cos(q4).*sin(q2)+ ...
  cos(q2).*sin(q4)).*sin(q5))+(-1).*(cos(q6).*(cos(q5).*((-1).*cos(q3).* ...
  cos(q4).*sin(q2)+cos(q2).*sin(q4))+sin(q2).*sin(q3).*sin(q5))+((-1).* ...
  cos(q2).*cos(q4)+(-1).*cos(q3).*sin(q2).*sin(q4)).*sin(q6)).*sin(q7))+(( ...
  -1).*cos(q6).*((-1).*cos(q2).*cos(q4)+(-1).*cos(q3).*sin(q2).*sin(q4))+( ...
  cos(q5).*((-1).*cos(q3).*cos(q4).*sin(q2)+cos(q2).*sin(q4))+sin(q2).* ...
  sin(q3).*sin(q5)).*sin(q6)).^(-1).*(cos(q7).*((-1).*cos(q3).*cos(q4).* ...
  sin(q2)+cos(q2).*sin(q4)).*sin(q5)+((-1).*cos(q5).*cos(q6).*(cos(q3).* ...
  cos(q4).*sin(q2)+(-1).*cos(q2).*sin(q4))+(-1).*(cos(q2).*cos(q4)+cos(q3) ...
  .*sin(q2).*sin(q4)).*sin(q6)).*sin(q7));

Jxe265 = ((-1).*cos(q6).*((-1).*cos(q2).* ...
  cos(q4)+(-1).*cos(q3).*sin(q2).*sin(q4))+(cos(q5).*((-1).*cos(q3).*cos( ...
  q4).*sin(q2)+cos(q2).*sin(q4))+sin(q2).*sin(q3).*sin(q5)).*sin(q6)).^( ...
  -1).*(cos(q7).*((-1).*cos(q5).*sin(q2).*sin(q3)+((-1).*cos(q3).*cos(q4) ...
  .*sin(q2)+cos(q2).*sin(q4)).*sin(q5))+(-1).*cos(q6).*((-1).*cos(q5).*(( ...
  -1).*cos(q3).*cos(q4).*sin(q2)+cos(q2).*sin(q4))+(-1).*sin(q2).*sin(q3) ...
  .*sin(q5)).*sin(q7))+(-2).*(cos(q5).*sin(q2).*sin(q3)+(-1).*((-1).*cos( ...
  q3).*cos(q4).*sin(q2)+cos(q2).*sin(q4)).*sin(q5)).*sin(q6).*((-1).*cos( ...
  q6).*((-1).*cos(q2).*cos(q4)+(-1).*cos(q3).*sin(q2).*sin(q4))+(cos(q5).* ...
  ((-1).*cos(q3).*cos(q4).*sin(q2)+cos(q2).*sin(q4))+sin(q2).*sin(q3).* ...
  sin(q5)).*sin(q6)).^(-2).*(cos(q7).*((-1).*cos(q5).*((-1).*cos(q3).*cos( ...
  q4).*sin(q2)+cos(q2).*sin(q4))+(-1).*sin(q2).*sin(q3).*sin(q5))+(-1).* ...
  cos(q6).*(cos(q5).*sin(q2).*sin(q3)+(-1).*((-1).*cos(q3).*cos(q4).*sin( ...
  q2)+cos(q2).*sin(q4)).*sin(q5)).*sin(q7))+(2.*(cos(q5).*sin(q2).*sin(q3) ...
  +(-1).*((-1).*cos(q3).*cos(q4).*sin(q2)+cos(q2).*sin(q4)).*sin(q5)).^2.* ...
  sin(q6).^2.*((-1).*cos(q6).*((-1).*cos(q2).*cos(q4)+(-1).*cos(q3).*sin( ...
  q2).*sin(q4))+(cos(q5).*((-1).*cos(q3).*cos(q4).*sin(q2)+cos(q2).*sin( ...
  q4))+sin(q2).*sin(q3).*sin(q5)).*sin(q6)).^(-3)+(-1).*((-1).*cos(q5).*(( ...
  -1).*cos(q3).*cos(q4).*sin(q2)+cos(q2).*sin(q4))+(-1).*sin(q2).*sin(q3) ...
  .*sin(q5)).*sin(q6).*((-1).*cos(q6).*((-1).*cos(q2).*cos(q4)+(-1).*cos( ...
  q3).*sin(q2).*sin(q4))+(cos(q5).*((-1).*cos(q3).*cos(q4).*sin(q2)+cos( ...
  q2).*sin(q4))+sin(q2).*sin(q3).*sin(q5)).*sin(q6)).^(-2)).*(cos(q7).*( ...
  cos(q5).*sin(q2).*sin(q3)+(-1).*((-1).*cos(q3).*cos(q4).*sin(q2)+cos(q2) ...
  .*sin(q4)).*sin(q5))+(-1).*(cos(q6).*(cos(q5).*((-1).*cos(q3).*cos(q4).* ...
  sin(q2)+cos(q2).*sin(q4))+sin(q2).*sin(q3).*sin(q5))+((-1).*cos(q2).* ...
  cos(q4)+(-1).*cos(q3).*sin(q2).*sin(q4)).*sin(q6)).*sin(q7));

Jxe266 = 2.*(cos(q6) ...
  .*(cos(q5).*((-1).*cos(q3).*cos(q4).*sin(q2)+cos(q2).*sin(q4))+sin(q2).* ...
  sin(q3).*sin(q5))+((-1).*cos(q2).*cos(q4)+(-1).*cos(q3).*sin(q2).*sin( ...
  q4)).*sin(q6)).*(cos(q6).*((-1).*cos(q2).*cos(q4)+(-1).*cos(q3).*sin(q2) ...
  .*sin(q4))+(-1).*(cos(q5).*((-1).*cos(q3).*cos(q4).*sin(q2)+cos(q2).* ...
  sin(q4))+sin(q2).*sin(q3).*sin(q5)).*sin(q6)).*((-1).*cos(q6).*((-1).* ...
  cos(q2).*cos(q4)+(-1).*cos(q3).*sin(q2).*sin(q4))+(cos(q5).*((-1).*cos( ...
  q3).*cos(q4).*sin(q2)+cos(q2).*sin(q4))+sin(q2).*sin(q3).*sin(q5)).*sin( ...
  q6)).^(-2).*sin(q7)+(cos(q6).*(cos(q5).*((-1).*cos(q3).*cos(q4).*sin(q2) ...
  +cos(q2).*sin(q4))+sin(q2).*sin(q3).*sin(q5))+((-1).*cos(q2).*cos(q4)+( ...
  -1).*cos(q3).*sin(q2).*sin(q4)).*sin(q6)).*((-1).*cos(q6).*((-1).*cos( ...
  q2).*cos(q4)+(-1).*cos(q3).*sin(q2).*sin(q4))+(cos(q5).*((-1).*cos(q3).* ...
  cos(q4).*sin(q2)+cos(q2).*sin(q4))+sin(q2).*sin(q3).*sin(q5)).*sin(q6)) ...
  .^(-1).*sin(q7)+(2.*(cos(q6).*(cos(q5).*((-1).*cos(q3).*cos(q4).*sin(q2) ...
  +cos(q2).*sin(q4))+sin(q2).*sin(q3).*sin(q5))+((-1).*cos(q2).*cos(q4)+( ...
  -1).*cos(q3).*sin(q2).*sin(q4)).*sin(q6)).^2.*((-1).*cos(q6).*((-1).* ...
  cos(q2).*cos(q4)+(-1).*cos(q3).*sin(q2).*sin(q4))+(cos(q5).*((-1).*cos( ...
  q3).*cos(q4).*sin(q2)+cos(q2).*sin(q4))+sin(q2).*sin(q3).*sin(q5)).*sin( ...
  q6)).^(-3)+(-1).*(cos(q6).*((-1).*cos(q2).*cos(q4)+(-1).*cos(q3).*sin( ...
  q2).*sin(q4))+(-1).*(cos(q5).*((-1).*cos(q3).*cos(q4).*sin(q2)+cos(q2).* ...
  sin(q4))+sin(q2).*sin(q3).*sin(q5)).*sin(q6)).*((-1).*cos(q6).*((-1).* ...
  cos(q2).*cos(q4)+(-1).*cos(q3).*sin(q2).*sin(q4))+(cos(q5).*((-1).*cos( ...
  q3).*cos(q4).*sin(q2)+cos(q2).*sin(q4))+sin(q2).*sin(q3).*sin(q5)).*sin( ...
  q6)).^(-2)).*(cos(q7).*(cos(q5).*sin(q2).*sin(q3)+(-1).*((-1).*cos(q3).* ...
  cos(q4).*sin(q2)+cos(q2).*sin(q4)).*sin(q5))+(-1).*(cos(q6).*(cos(q5).*( ...
  (-1).*cos(q3).*cos(q4).*sin(q2)+cos(q2).*sin(q4))+sin(q2).*sin(q3).*sin( ...
  q5))+((-1).*cos(q2).*cos(q4)+(-1).*cos(q3).*sin(q2).*sin(q4)).*sin(q6)) ...
  .*sin(q7));

Jxe267 = ((-1).*cos(q6).*((-1).*cos(q2).*cos(q4)+(-1).*cos(q3).*sin( ...
  q2).*sin(q4))+(cos(q5).*((-1).*cos(q3).*cos(q4).*sin(q2)+cos(q2).*sin( ...
  q4))+sin(q2).*sin(q3).*sin(q5)).*sin(q6)).^(-1).*((-1).*cos(q7).*(cos( ...
  q5).*sin(q2).*sin(q3)+(-1).*((-1).*cos(q3).*cos(q4).*sin(q2)+cos(q2).* ...
  sin(q4)).*sin(q5))+(cos(q6).*(cos(q5).*((-1).*cos(q3).*cos(q4).*sin(q2)+ ...
  cos(q2).*sin(q4))+sin(q2).*sin(q3).*sin(q5))+((-1).*cos(q2).*cos(q4)+( ...
  -1).*cos(q3).*sin(q2).*sin(q4)).*sin(q6)).*sin(q7));


Jxe2 = [Jxe211, Jxe212, Jxe213, Jxe214, Jxe215, Jxe216, Jxe217;
       Jxe221, Jxe222, Jxe223, Jxe224, Jxe225, Jxe226, Jxe227;
       Jxe231, Jxe232, Jxe233, Jxe234, Jxe235, Jxe236, Jxe237;
       Jxe241, Jxe242, Jxe243, Jxe244, Jxe245, Jxe246, Jxe247;
       Jxe251, Jxe252, Jxe253, Jxe254, Jxe255, Jxe256, Jxe257;
       Jxe261, Jxe262, Jxe263, Jxe264, Jxe265, Jxe266, Jxe267];


   
   
   
JxePseudoInv  = KUKAanaJacPseudoInv(Jxe);
%Jxe2PseudoInv = KUKAanaJacPseudoInv(Jxe2);




vecPosDes = [vecPosDes_, rpyDes_(1), rpyDes_(2), rpyDes_(3)];
vecVelDes = [vecVelDes_, 0, 0, 0]';
vecAccDes = [vecAccDes_, 0, 0, 0]';

qDDot0 = [0,0,0,0,0,0,0];

vecVelReal = Jxe * vecJointVelReal_;

vecJointAcc = JxePseudoInv * (vecAccDes + KAnaJacD_* (vecVelDes - vecVelReal) + ... 
              KAnaJacP_ * (vecPosDes - vecPosReal_)' - Jxe2 * vecJointVelReal_) + (eye(7) - JxePseudoInv*Jxe)*qDDot0';
vecJointVel = transpose(Jxe) * KAnaJacP_ * (vecPosDes - vecPosReal_)';

vecJointPos = vecJointPosDes_;
end



function [J_T] = KUKAanaJacPseudoInv(Jxe_)


J_T = transpose(Jxe_)*inv(Jxe_*Jxe_');

end
